simulink model "model"  (R2016a)
(part 9 of 11)

  Dellmensingen___Niederstotzingen_CN_31105067_380000_CN_41389594_380000/RConn3 -- T_41389594_380000;220000;110000_Umspannwerk_Dellmensingen/LConn3 -- 380_kV_CN_26260052_380000_CN_41389594_380000/LConn3 -- _CN_85523877_380000_CN_41389594_380000/RConn3 -- Dellmensingen___Obermooweiler;Dellmensingen_Ost_CN_41389594_380000_CN_31131320_380000/LConn3
  T_130794504_220000;110000_Lübeck/LConn1 -- _CN_130794504_220000_CN_28008024_220000/LConn1
  T_130794504_220000;110000_Lübeck/LConn2 -- _CN_130794504_220000_CN_28008024_220000/LConn2
  T_130794504_220000;110000_Lübeck/LConn3 -- _CN_130794504_220000_CN_28008024_220000/LConn3
  _CN_130794504_220000_CN_28008024_220000/RConn1 -- T_28008024_220000;110000;30000_Hamburg_Nord/LConn1 -- _CN_29344008_220000_CN_28008024_220000/RConn1 -- 202_UW_HH_Nord_UW_Itzehoe_West_CN_60032354_220000_CN_28008024_220000/LConn1 -- _CN_28008024_220000_CN_33148774_220000/LConn1 -- _CN_22720647_220000_CN_28008024_220000/LConn1
  _CN_130794504_220000_CN_28008024_220000/RConn2 -- T_28008024_220000;110000;30000_Hamburg_Nord/LConn2 -- _CN_29344008_220000_CN_28008024_220000/RConn2 -- 202_UW_HH_Nord_UW_Itzehoe_West_CN_60032354_220000_CN_28008024_220000/LConn2 -- _CN_28008024_220000_CN_33148774_220000/LConn2 -- _CN_22720647_220000_CN_28008024_220000/LConn2
  _CN_130794504_220000_CN_28008024_220000/RConn3 -- T_28008024_220000;110000;30000_Hamburg_Nord/LConn3 -- _CN_29344008_220000_CN_28008024_220000/RConn3 -- 202_UW_HH_Nord_UW_Itzehoe_West_CN_60032354_220000_CN_28008024_220000/LConn3 -- _CN_28008024_220000_CN_33148774_220000/LConn3 -- _CN_22720647_220000_CN_28008024_220000/LConn3
  543_CN_32063539_380000_CN_32062544_380000/LConn1 -- T_32063539_380000_Bentwisch_HGÜ/LConn1 -- 546_CN_32063539_380000_CN26389159/LConn1
  543_CN_32063539_380000_CN_32062544_380000/LConn2 -- T_32063539_380000_Bentwisch_HGÜ/LConn2 -- 546_CN_32063539_380000_CN26389159/LConn2
  543_CN_32063539_380000_CN_32062544_380000/LConn3 -- T_32063539_380000_Bentwisch_HGÜ/LConn3 -- 546_CN_32063539_380000_CN26389159/LConn3
  543_CN_32063539_380000_CN_32062544_380000/RConn1 -- T_32062544_380000;220000_Güstrow/LConn1 -- 514_CN_59707532_380000_CN_32062544_380000/LConn1 -- 419_Krümmel___Görries_CN_30040568_380000_CN_32062544_380000/LConn1
  543_CN_32063539_380000_CN_32062544_380000/RConn2 -- T_32062544_380000;220000_Güstrow/LConn2 -- 514_CN_59707532_380000_CN_32062544_380000/LConn2 -- 419_Krümmel___Görries_CN_30040568_380000_CN_32062544_380000/LConn2
  543_CN_32063539_380000_CN_32062544_380000/RConn3 -- T_32062544_380000;220000_Güstrow/LConn3 -- 514_CN_59707532_380000_CN_32062544_380000/LConn3 -- 419_Krümmel___Görries_CN_30040568_380000_CN_32062544_380000/LConn3
  G_26389159_Kraftwerk_Rostock/RConn1 -- 546_CN_32063539_380000_CN26389159/RConn1
  G_26389159_Kraftwerk_Rostock/RConn2 -- 546_CN_32063539_380000_CN26389159/RConn2
  G_26389159_Kraftwerk_Rostock/RConn3 -- 546_CN_32063539_380000_CN26389159/RConn3
  Grafenrheinfeld___Eltmann;Eltmann___Redwitz_CN_24758329_380000_CN_108797675_380000/LConn1 -- T_24758329_380000;110000_Umspannwerk_Eltmann/LConn1 -- Grafenrheinfeld___Eltmann;Eltmann___Redwitz_CN_24758329_380000_CN_28613721_380000/LConn1 -- Grafenrheinfeld___Eltmann;Eltmann___Redwitz_CN_24758329_380000_CN_24757392_380000/LConn1 -- Grafenrheinfeld___Eltmann;Eltmann___Redwitz_CN_24758329_380000_CN_24757833_380000/LConn1 -- Grafenrheinfeld___Eltmann;Eltmann___Redwitz_CN_24758329_380000_CN_24715381_380000/LConn1 -- Grafenrheinfeld___Eltmann;Eltmann___Redwitz_CN_24758329_380000_CN_24705761_380000/LConn1
  Grafenrheinfeld___Eltmann;Eltmann___Redwitz_CN_24758329_380000_CN_108797675_380000/LConn2 -- T_24758329_380000;110000_Umspannwerk_Eltmann/LConn2 -- Grafenrheinfeld___Eltmann;Eltmann___Redwitz_CN_24758329_380000_CN_28613721_380000/LConn2 -- Grafenrheinfeld___Eltmann;Eltmann___Redwitz_CN_24758329_380000_CN_24757392_380000/LConn2 -- Grafenrheinfeld___Eltmann;Eltmann___Redwitz_CN_24758329_380000_CN_24757833_380000/LConn2 -- Grafenrheinfeld___Eltmann;Eltmann___Redwitz_CN_24758329_380000_CN_24715381_380000/LConn2 -- Grafenrheinfeld___Eltmann;Eltmann___Redwitz_CN_24758329_380000_CN_24705761_380000/LConn2
  Grafenrheinfeld___Eltmann;Eltmann___Redwitz_CN_24758329_380000_CN_108797675_380000/LConn3 -- T_24758329_380000;110000_Umspannwerk_Eltmann/LConn3 -- Grafenrheinfeld___Eltmann;Eltmann___Redwitz_CN_24758329_380000_CN_28613721_380000/LConn3 -- Grafenrheinfeld___Eltmann;Eltmann___Redwitz_CN_24758329_380000_CN_24757392_380000/LConn3 -- Grafenrheinfeld___Eltmann;Eltmann___Redwitz_CN_24758329_380000_CN_24757833_380000/LConn3 -- Grafenrheinfeld___Eltmann;Eltmann___Redwitz_CN_24758329_380000_CN_24715381_380000/LConn3 -- Grafenrheinfeld___Eltmann;Eltmann___Redwitz_CN_24758329_380000_CN_24705761_380000/LConn3
  Grafenrheinfeld___Eltmann;Eltmann___Redwitz_CN_24758329_380000_CN_108797675_380000/RConn1 -- T_108797675_380000_Grafenrheinfeld/LConn1 -- _CN_24715381_380000_CN_108797675_380000/LConn1 -- _CN_145002769_380000_CN_108797675_380000/LConn1 -- _CN_24705761_380000_CN_108797675_380000/LConn1 -- AS_GKRO;GKRO_GR_I;DIP_GKB_I;_II_CN_42410916_380000_CN_108797675_380000/LConn1
  Grafenrheinfeld___Eltmann;Eltmann___Redwitz_CN_24758329_380000_CN_108797675_380000/RConn2 -- T_108797675_380000_Grafenrheinfeld/LConn2 -- _CN_24715381_380000_CN_108797675_380000/LConn2 -- _CN_145002769_380000_CN_108797675_380000/LConn2 -- _CN_24705761_380000_CN_108797675_380000/LConn2 -- AS_GKRO;GKRO_GR_I;DIP_GKB_I;_II_CN_42410916_380000_CN_108797675_380000/LConn2
  Grafenrheinfeld___Eltmann;Eltmann___Redwitz_CN_24758329_380000_CN_108797675_380000/RConn3 -- T_108797675_380000_Grafenrheinfeld/LConn3 -- _CN_24715381_380000_CN_108797675_380000/LConn3 -- _CN_145002769_380000_CN_108797675_380000/LConn3 -- _CN_24705761_380000_CN_108797675_380000/LConn3 -- AS_GKRO;GKRO_GR_I;DIP_GKB_I;_II_CN_42410916_380000_CN_108797675_380000/LConn3
  Grafenrheinfeld___Eltmann;Eltmann___Redwitz_CN_24758329_380000_CN_24715381_380000/RConn1 -- T_24715381_380000;220000;110000_Umspannwerk_Bergrheinfeld/LConn1 -- _CN_24715381_380000_CN_108797675_380000/RConn1
  Grafenrheinfeld___Eltmann;Eltmann___Redwitz_CN_24758329_380000_CN_24715381_380000/RConn2 -- T_24715381_380000;220000;110000_Umspannwerk_Bergrheinfeld/LConn2 -- _CN_24715381_380000_CN_108797675_380000/RConn2
  Grafenrheinfeld___Eltmann;Eltmann___Redwitz_CN_24758329_380000_CN_24715381_380000/RConn3 -- T_24715381_380000;220000;110000_Umspannwerk_Bergrheinfeld/LConn3 -- _CN_24715381_380000_CN_108797675_380000/RConn3
  Grafenrheinfeld___Eltmann;Eltmann___Redwitz_CN_24758329_380000_CN_24705761_380000/RConn1 -- T_24705761_380000;220000;110000_Umspannwerk_Raitersaich/LConn1 -- Irsching___Raitersaich_CN_24705761_380000_CN_24768051_380000/LConn1 -- _CN_24705761_380000_CN_108797675_380000/RConn1
  Grafenrheinfeld___Eltmann;Eltmann___Redwitz_CN_24758329_380000_CN_24705761_380000/RConn2 -- T_24705761_380000;220000;110000_Umspannwerk_Raitersaich/LConn2 -- Irsching___Raitersaich_CN_24705761_380000_CN_24768051_380000/LConn2 -- _CN_24705761_380000_CN_108797675_380000/RConn2
  Grafenrheinfeld___Eltmann;Eltmann___Redwitz_CN_24758329_380000_CN_24705761_380000/RConn3 -- T_24705761_380000;220000;110000_Umspannwerk_Raitersaich/LConn3 -- Irsching___Raitersaich_CN_24705761_380000_CN_24768051_380000/LConn3 -- _CN_24705761_380000_CN_108797675_380000/RConn3
  T_28613721_380000;110000_Kriegenbrunn/LConn1 -- Grafenrheinfeld___Eltmann;Eltmann___Redwitz_CN_24758329_380000_CN_28613721_380000/RConn1
  T_28613721_380000;110000_Kriegenbrunn/LConn2 -- Grafenrheinfeld___Eltmann;Eltmann___Redwitz_CN_24758329_380000_CN_28613721_380000/RConn2
  T_28613721_380000;110000_Kriegenbrunn/LConn3 -- Grafenrheinfeld___Eltmann;Eltmann___Redwitz_CN_24758329_380000_CN_28613721_380000/RConn3
  Grafenrheinfeld___Eltmann;Eltmann___Redwitz_CN_24758329_380000_CN_24757392_380000/RConn1 -- T_24757392_380000;110000_Umspannwerk_Redwitz/LConn1 -- Etzenricht___Mechlenreuth___Redwitz_CN_93341407_380000_CN_24757392_380000/LConn1 -- _CN_128277645_380000_CN_24757392_380000/LConn1 -- Altenfeld___Redwitz_CN_149256409_380000_CN_24757392_380000/LConn1
  Grafenrheinfeld___Eltmann;Eltmann___Redwitz_CN_24758329_380000_CN_24757392_380000/RConn2 -- T_24757392_380000;110000_Umspannwerk_Redwitz/LConn2 -- Etzenricht___Mechlenreuth___Redwitz_CN_93341407_380000_CN_24757392_380000/LConn2 -- _CN_128277645_380000_CN_24757392_380000/LConn2 -- Altenfeld___Redwitz_CN_149256409_380000_CN_24757392_380000/LConn2
  Grafenrheinfeld___Eltmann;Eltmann___Redwitz_CN_24758329_380000_CN_24757392_380000/RConn3 -- T_24757392_380000;110000_Umspannwerk_Redwitz/LConn3 -- Etzenricht___Mechlenreuth___Redwitz_CN_93341407_380000_CN_24757392_380000/LConn3 -- _CN_128277645_380000_CN_24757392_380000/LConn3 -- Altenfeld___Redwitz_CN_149256409_380000_CN_24757392_380000/LConn3
  T_24757833_380000_Umspannwerk_Oberhaid/LConn1 -- Grafenrheinfeld___Eltmann;Eltmann___Redwitz_CN_24758329_380000_CN_24757833_380000/RConn1
  T_24757833_380000_Umspannwerk_Oberhaid/LConn2 -- Grafenrheinfeld___Eltmann;Eltmann___Redwitz_CN_24758329_380000_CN_24757833_380000/RConn2
  T_24757833_380000_Umspannwerk_Oberhaid/LConn3 -- Grafenrheinfeld___Eltmann;Eltmann___Redwitz_CN_24758329_380000_CN_24757833_380000/RConn3
  220kV_Itterbach_West_CN_87767098_220000_CN_113546939_220000/LConn1 -- T_87767098_220000_Station_Mettmann/LConn1 -- 220kV_Itterbach_West_CN_87767098_220000_CN_23192640_220000/LConn1 -- 220kV_Itterbach_West_CN_87767098_220000_CN_49577401_220000/LConn1 -- 220kV_Itterbach_West_CN_87767098_220000_CN_23140544_220000/LConn1 -- 220kV_Itterbach_West_CN_87767098_220000_CN_22761839_220000/LConn1
  220kV_Itterbach_West_CN_87767098_220000_CN_113546939_220000/LConn2 -- T_87767098_220000_Station_Mettmann/LConn2 -- 220kV_Itterbach_West_CN_87767098_220000_CN_23192640_220000/LConn2 -- 220kV_Itterbach_West_CN_87767098_220000_CN_49577401_220000/LConn2 -- 220kV_Itterbach_West_CN_87767098_220000_CN_23140544_220000/LConn2 -- 220kV_Itterbach_West_CN_87767098_220000_CN_22761839_220000/LConn2
  220kV_Itterbach_West_CN_87767098_220000_CN_113546939_220000/LConn3 -- T_87767098_220000_Station_Mettmann/LConn3 -- 220kV_Itterbach_West_CN_87767098_220000_CN_23192640_220000/LConn3 -- 220kV_Itterbach_West_CN_87767098_220000_CN_49577401_220000/LConn3 -- 220kV_Itterbach_West_CN_87767098_220000_CN_23140544_220000/LConn3 -- 220kV_Itterbach_West_CN_87767098_220000_CN_22761839_220000/LConn3
  220kV_Itterbach_West_CN_87767098_220000_CN_113546939_220000/RConn1 -- T_113546939_380000;220000_Station_Eiberg/RConn1 -- _CN_66038431_220000_CN_113546939_220000/LConn1 -- L_113546939/LConn1 -- 220kV_Polsum_Süd_CN_29077623_220000_CN_113546939_220000/LConn1
  220kV_Itterbach_West_CN_87767098_220000_CN_113546939_220000/RConn2 -- T_113546939_380000;220000_Station_Eiberg/RConn2 -- _CN_66038431_220000_CN_113546939_220000/LConn2 -- L_113546939/LConn2 -- 220kV_Polsum_Süd_CN_29077623_220000_CN_113546939_220000/LConn2
  220kV_Itterbach_West_CN_87767098_220000_CN_113546939_220000/RConn3 -- T_113546939_380000;220000_Station_Eiberg/RConn3 -- _CN_66038431_220000_CN_113546939_220000/LConn3 -- L_113546939/LConn3 -- 220kV_Polsum_Süd_CN_29077623_220000_CN_113546939_220000/LConn3
  T_23192640_220000;110000_Station_Reisholz/LConn1 -- 220kV_Itterbach_West_CN_87767098_220000_CN_23192640_220000/RConn1
  T_23192640_220000;110000_Station_Reisholz/LConn2 -- 220kV_Itterbach_West_CN_87767098_220000_CN_23192640_220000/RConn2
  T_23192640_220000;110000_Station_Reisholz/LConn3 -- 220kV_Itterbach_West_CN_87767098_220000_CN_23192640_220000/RConn3
  220kV_Itterbach_West_CN_87767098_220000_CN_49577401_220000/RConn1 -- T_49577401_220000;110000_Station_Sankt_Peter_220_kV/LConn1 -- 220_kV_Frixheim_Süd;_Zons_Nord_CN_27919734_220000_CN_49577401_220000/LConn1 -- 220_kV_Frimmersdorf_5e;_Zons_Nord_CN_49577401_220000_CN_31762305_220000/LConn1
  220kV_Itterbach_West_CN_87767098_220000_CN_49577401_220000/RConn2 -- T_49577401_220000;110000_Station_Sankt_Peter_220_kV/LConn2 -- 220_kV_Frixheim_Süd;_Zons_Nord_CN_27919734_220000_CN_49577401_220000/LConn2 -- 220_kV_Frimmersdorf_5e;_Zons_Nord_CN_49577401_220000_CN_31762305_220000/LConn2
  220kV_Itterbach_West_CN_87767098_220000_CN_49577401_220000/RConn3 -- T_49577401_220000;110000_Station_Sankt_Peter_220_kV/LConn3 -- 220_kV_Frixheim_Süd;_Zons_Nord_CN_27919734_220000_CN_49577401_220000/LConn3 -- 220_kV_Frimmersdorf_5e;_Zons_Nord_CN_49577401_220000_CN_31762305_220000/LConn3
  T_23140544_220000;110000_Station_Eller/LConn1 -- 220kV_Itterbach_West_CN_87767098_220000_CN_23140544_220000/RConn1
  T_23140544_220000;110000_Station_Eller/LConn2 -- 220kV_Itterbach_West_CN_87767098_220000_CN_23140544_220000/RConn2
  T_23140544_220000;110000_Station_Eller/LConn3 -- 220kV_Itterbach_West_CN_87767098_220000_CN_23140544_220000/RConn3
  220kV_Itterbach_West_CN_87767098_220000_CN_22761839_220000/RConn1 -- T_22761839_380000;220000;110000_Station_Opladen/RConn1 -- 220_kV_Niederaußem_4d;_Wiesdorf_Ltg__CN_22761839_220000_CN_24839976_220000/LConn1 -- 220_kV_Niederaußem_4d;_Wiesdorf_Ltg__CN_22761839_220000_CN24840439/LConn1 -- 220_kV_Niederaußem_4d;_Wiesdorf_Ltg__CN_22761839_220000_CN_22764922_220000/LConn1 -- 220_kV_Dünnwald_Ost|West_CN_22761839_220000_CN_27871140_220000/LConn1 -- L_22761839/LConn1 -- 220_kV_Bigge_Ost|West_CN_22761839_220000_CN_24667346_220000/LConn1 -- 220_kV_Bigge_Ost|West_CN_22761839_220000_CN_51940126_220000/LConn1 -- 220_kV_Bigge_Ost|West_CN_22761839_220000_CN_132814303_220000/LConn1 -- 220_kV_Niederaußem_4d;_Wiesdorf_Ltg__CN_22761839_220000_CN_22761692_220000/LConn1
  220kV_Itterbach_West_CN_87767098_220000_CN_22761839_220000/RConn2 -- T_22761839_380000;220000;110000_Station_Opladen/RConn2 -- 220_kV_Niederaußem_4d;_Wiesdorf_Ltg__CN_22761839_220000_CN_24839976_220000/LConn2 -- 220_kV_Niederaußem_4d;_Wiesdorf_Ltg__CN_22761839_220000_CN24840439/LConn2 -- 220_kV_Niederaußem_4d;_Wiesdorf_Ltg__CN_22761839_220000_CN_22764922_220000/LConn2 -- 220_kV_Dünnwald_Ost|West_CN_22761839_220000_CN_27871140_220000/LConn2 -- L_22761839/LConn2 -- 220_kV_Bigge_Ost|West_CN_22761839_220000_CN_24667346_220000/LConn2 -- 220_kV_Bigge_Ost|West_CN_22761839_220000_CN_51940126_220000/LConn2 -- 220_kV_Bigge_Ost|West_CN_22761839_220000_CN_132814303_220000/LConn2 -- 220_kV_Niederaußem_4d;_Wiesdorf_Ltg__CN_22761839_220000_CN_22761692_220000/LConn2
  220kV_Itterbach_West_CN_87767098_220000_CN_22761839_220000/RConn3 -- T_22761839_380000;220000;110000_Station_Opladen/RConn3 -- 220_kV_Niederaußem_4d;_Wiesdorf_Ltg__CN_22761839_220000_CN_24839976_220000/LConn3 -- 220_kV_Niederaußem_4d;_Wiesdorf_Ltg__CN_22761839_220000_CN24840439/LConn3 -- 220_kV_Niederaußem_4d;_Wiesdorf_Ltg__CN_22761839_220000_CN_22764922_220000/LConn3 -- 220_kV_Dünnwald_Ost|West_CN_22761839_220000_CN_27871140_220000/LConn3 -- L_22761839/LConn3 -- 220_kV_Bigge_Ost|West_CN_22761839_220000_CN_24667346_220000/LConn3 -- 220_kV_Bigge_Ost|West_CN_22761839_220000_CN_51940126_220000/LConn3 -- 220_kV_Bigge_Ost|West_CN_22761839_220000_CN_132814303_220000/LConn3 -- 220_kV_Niederaußem_4d;_Wiesdorf_Ltg__CN_22761839_220000_CN_22761692_220000/LConn3
  _CN_88916034_380000_CN_35954395_380000/LConn1 -- T_88916034_380000;220000_Lastverteilung_Schaltanlage_Kühmoos/LConn1 -- _CN_88916034_380000_CN_25306752_380000/LConn1 -- _CN_88916034_380000_CN_31367940_380000/LConn1 -- _CN_88916034_380000_CN_202865177_380000/LConn1 -- _CN_88916034_380000_CN_88901626_380000/LConn1 -- _CN_88916034_380000_CN_242756113_380000/LConn1 -- _CN_88916034_380000_CN_152261133_380000/LConn1 -- _CN_88916034_380000_CN_42736239_380000/LConn1 -- _CN_88916034_380000_CN_42049947_380000/LConn1
  _CN_88916034_380000_CN_35954395_380000/LConn2 -- T_88916034_380000;220000_Lastverteilung_Schaltanlage_Kühmoos/LConn2 -- _CN_88916034_380000_CN_25306752_380000/LConn2 -- _CN_88916034_380000_CN_31367940_380000/LConn2 -- _CN_88916034_380000_CN_202865177_380000/LConn2 -- _CN_88916034_380000_CN_88901626_380000/LConn2 -- _CN_88916034_380000_CN_242756113_380000/LConn2 -- _CN_88916034_380000_CN_152261133_380000/LConn2 -- _CN_88916034_380000_CN_42736239_380000/LConn2 -- _CN_88916034_380000_CN_42049947_380000/LConn2
  _CN_88916034_380000_CN_35954395_380000/LConn3 -- T_88916034_380000;220000_Lastverteilung_Schaltanlage_Kühmoos/LConn3 -- _CN_88916034_380000_CN_25306752_380000/LConn3 -- _CN_88916034_380000_CN_31367940_380000/LConn3 -- _CN_88916034_380000_CN_202865177_380000/LConn3 -- _CN_88916034_380000_CN_88901626_380000/LConn3 -- _CN_88916034_380000_CN_242756113_380000/LConn3 -- _CN_88916034_380000_CN_152261133_380000/LConn3 -- _CN_88916034_380000_CN_42736239_380000/LConn3 -- _CN_88916034_380000_CN_42049947_380000/LConn3
  T_35954395_380000;110000_Umspannwerk_Trossingen/LConn1 -- _CN_88916034_380000_CN_35954395_380000/RConn1
  T_35954395_380000;110000_Umspannwerk_Trossingen/LConn2 -- _CN_88916034_380000_CN_35954395_380000/RConn2
  T_35954395_380000;110000_Umspannwerk_Trossingen/LConn3 -- _CN_88916034_380000_CN_35954395_380000/RConn3
  _CN_88916034_380000_CN_42736239_380000/RConn1 -- T_42736239_380000_EnBW_Umspannwerk_Engstlatt/LConn1 -- PULVE_OBJTT_ENGST_380_kV;_OBJTT_ENGST_380_kV;_TRSNG_WDLNG_220_kV_CN_42736239_380000_CN_26814283_380000/LConn1
  _CN_88916034_380000_CN_42736239_380000/RConn2 -- T_42736239_380000_EnBW_Umspannwerk_Engstlatt/LConn2 -- PULVE_OBJTT_ENGST_380_kV;_OBJTT_ENGST_380_kV;_TRSNG_WDLNG_220_kV_CN_42736239_380000_CN_26814283_380000/LConn2
  _CN_88916034_380000_CN_42736239_380000/RConn3 -- T_42736239_380000_EnBW_Umspannwerk_Engstlatt/LConn3 -- PULVE_OBJTT_ENGST_380_kV;_OBJTT_ENGST_380_kV;_TRSNG_WDLNG_220_kV_CN_42736239_380000_CN_26814283_380000/LConn3
  T_42049947_380000;110000_Umspannwerk_Villingen/LConn1 -- _CN_88916034_380000_CN_42049947_380000/RConn1
  T_42049947_380000;110000_Umspannwerk_Villingen/LConn2 -- _CN_88916034_380000_CN_42049947_380000/RConn2
  T_42049947_380000;110000_Umspannwerk_Villingen/LConn3 -- _CN_88916034_380000_CN_42049947_380000/RConn3
  T_88901626_380000;110000_Schwörstadt/LConn1 -- _CN_88916034_380000_CN_88901626_380000/RConn1
  T_88901626_380000;110000_Schwörstadt/LConn2 -- _CN_88916034_380000_CN_88901626_380000/RConn2
  T_88901626_380000;110000_Schwörstadt/LConn3 -- _CN_88916034_380000_CN_88901626_380000/RConn3
  T_242756113_380000;220000;110000_380_kV_Umspannwerk_Eichstetten/LConn1 -- _CN_88916034_380000_CN_242756113_380000/RConn1
  T_242756113_380000;220000;110000_380_kV_Umspannwerk_Eichstetten/LConn2 -- _CN_88916034_380000_CN_242756113_380000/RConn2
  T_242756113_380000;220000;110000_380_kV_Umspannwerk_Eichstetten/LConn3 -- _CN_88916034_380000_CN_242756113_380000/RConn3
  _CN_88916034_380000_CN_152261133_380000/RConn1 -- T_152261133_380000;220000;110000_Karlsruhe_Daxlanden/LConn1 -- _CN_152261133_380000_CN_149987048_380000/LConn1 -- _CN_152261133_380000_CN_54359256_380000/LConn1 -- _CN_152261133_380000_CN_152018146_380000/LConn1 -- _CN_152261133_380000_CN161909939/LConn1 -- 7563_CN_152261133_380000_CN_272646943_380000/LConn1 -- 7564_CN_152261133_380000_CN_194446360_380000/LConn1
  _CN_88916034_380000_CN_152261133_380000/RConn2 -- T_152261133_380000;220000;110000_Karlsruhe_Daxlanden/LConn2 -- _CN_152261133_380000_CN_149987048_380000/LConn2 -- _CN_152261133_380000_CN_54359256_380000/LConn2 -- _CN_152261133_380000_CN_152018146_380000/LConn2 -- _CN_152261133_380000_CN161909939/LConn2 -- 7563_CN_152261133_380000_CN_272646943_380000/LConn2 -- 7564_CN_152261133_380000_CN_194446360_380000/LConn2
  _CN_88916034_380000_CN_152261133_380000/RConn3 -- T_152261133_380000;220000;110000_Karlsruhe_Daxlanden/LConn3 -- _CN_152261133_380000_CN_149987048_380000/LConn3 -- _CN_152261133_380000_CN_54359256_380000/LConn3 -- _CN_152261133_380000_CN_152018146_380000/LConn3 -- _CN_152261133_380000_CN161909939/LConn3 -- 7563_CN_152261133_380000_CN_272646943_380000/LConn3 -- 7564_CN_152261133_380000_CN_194446360_380000/LConn3
  _CN_88916034_380000_CN_25306752_380000/RConn1 -- T_25306752_380000;220000;110000_Umspannwerk_Herbertingen/LConn1 -- Herbertingen___Grünkraut_CN_25306752_380000_CN_31131325_380000/LConn1
  _CN_88916034_380000_CN_25306752_380000/RConn2 -- T_25306752_380000;220000;110000_Umspannwerk_Herbertingen/LConn2 -- Herbertingen___Grünkraut_CN_25306752_380000_CN_31131325_380000/LConn2
  _CN_88916034_380000_CN_25306752_380000/RConn3 -- T_25306752_380000;220000;110000_Umspannwerk_Herbertingen/LConn3 -- Herbertingen___Grünkraut_CN_25306752_380000_CN_31131325_380000/LConn3
  T_31367940_380000;220000;110000_Tiengen/LConn1 -- _CN_88916034_380000_CN_31367940_380000/RConn1
  T_31367940_380000;220000;110000_Tiengen/LConn2 -- _CN_88916034_380000_CN_31367940_380000/RConn2
  T_31367940_380000;220000;110000_Tiengen/LConn3 -- _CN_88916034_380000_CN_31367940_380000/RConn3
  _CN_88916034_220000_CN_202865176_220000/LConn1 -- T_88916034_380000;220000_Lastverteilung_Schaltanlage_Kühmoos/RConn1 -- L_88916034/LConn1
  _CN_88916034_220000_CN_202865176_220000/LConn2 -- T_88916034_380000;220000_Lastverteilung_Schaltanlage_Kühmoos/RConn2 -- L_88916034/LConn2
  _CN_88916034_220000_CN_202865176_220000/LConn3 -- T_88916034_380000;220000_Lastverteilung_Schaltanlage_Kühmoos/RConn3 -- L_88916034/LConn3
  _CN_88916034_220000_CN_202865176_220000/RConn1 -- T_202865176_220000_/LConn1 -- Öldruckkabel_CN_202865176_220000_CN129989100/LConn1
  _CN_88916034_220000_CN_202865176_220000/RConn2 -- T_202865176_220000_/LConn2 -- Öldruckkabel_CN_202865176_220000_CN129989100/LConn2
  _CN_88916034_220000_CN_202865176_220000/RConn3 -- T_202865176_220000_/LConn3 -- Öldruckkabel_CN_202865176_220000_CN129989100/LConn3
  T_202865177_380000_Kabelanfang_PSP_Wehr/LConn1 -- _CN_88916034_380000_CN_202865177_380000/RConn1
  T_202865177_380000_Kabelanfang_PSP_Wehr/LConn2 -- _CN_88916034_380000_CN_202865177_380000/RConn2
  T_202865177_380000_Kabelanfang_PSP_Wehr/LConn3 -- _CN_88916034_380000_CN_202865177_380000/RConn3
  _CN_32151621_220000_CN_39011884_220000/LConn1 -- T_32151621_220000;110000_220_kV_Umspannwerk_Kuppenheim/LConn1 -- _CN_32151621_220000_CN_146962222_220000/LConn1 -- _CN_32151621_220000_CN_152261133_220000/LConn1
  _CN_32151621_220000_CN_39011884_220000/LConn2 -- T_32151621_220000;110000_220_kV_Umspannwerk_Kuppenheim/LConn2 -- _CN_32151621_220000_CN_146962222_220000/LConn2 -- _CN_32151621_220000_CN_152261133_220000/LConn2
  _CN_32151621_220000_CN_39011884_220000/LConn3 -- T_32151621_220000;110000_220_kV_Umspannwerk_Kuppenheim/LConn3 -- _CN_32151621_220000_CN_146962222_220000/LConn3 -- _CN_32151621_220000_CN_152261133_220000/LConn3
  T_39011884_220000;110000_Bühl/LConn1 -- _CN_32151621_220000_CN_39011884_220000/RConn1
  T_39011884_220000;110000_Bühl/LConn2 -- _CN_32151621_220000_CN_39011884_220000/RConn2
  T_39011884_220000;110000_Bühl/LConn3 -- _CN_32151621_220000_CN_39011884_220000/RConn3
  _CN_32151621_220000_CN_146962222_220000/RConn1 -- T_146962222_220000;110000_Umspannwerk_Weier/LConn1 -- _CN_87653464_220000_CN_146962222_220000/LConn1
  _CN_32151621_220000_CN_146962222_220000/RConn2 -- T_146962222_220000;110000_Umspannwerk_Weier/LConn2 -- _CN_87653464_220000_CN_146962222_220000/LConn2
  _CN_32151621_220000_CN_146962222_220000/RConn3 -- T_146962222_220000;110000_Umspannwerk_Weier/LConn3 -- _CN_87653464_220000_CN_146962222_220000/LConn3
  _CN_32151621_220000_CN_152261133_220000/RConn1 -- T_152261133_380000;220000;110000_Karlsruhe_Daxlanden/RConn1 -- Daxlanden___Mühlburg_CN_32731290_220000_CN_152261133_220000/LConn1 -- _CN_152261133_220000_CN_207248812_220000/RConn1 -- _CN_152261133_220000_CN_163093653_220000/LConn1 -- _CN_152261133_220000_CN_160929097_220000/LConn1 -- _CN_152261133_220000_CN_154729020_220000/LConn1 -- _CN_152261133_220000_CN_32966636_220000/LConn1 -- _CN_152261133_220000_CN_32725957_220000/LConn1 -- L_152261133/LConn1 -- 220_kV_Kondelwald;_220kV_Wengerohr_CN_66764943_220000_CN_152261133_220000/LConn1
  _CN_32151621_220000_CN_152261133_220000/RConn2 -- T_152261133_380000;220000;110000_Karlsruhe_Daxlanden/RConn2 -- Daxlanden___Mühlburg_CN_32731290_220000_CN_152261133_220000/LConn2 -- _CN_152261133_220000_CN_207248812_220000/RConn2 -- _CN_152261133_220000_CN_163093653_220000/LConn2 -- _CN_152261133_220000_CN_160929097_220000/LConn2 -- _CN_152261133_220000_CN_154729020_220000/LConn2 -- _CN_152261133_220000_CN_32966636_220000/LConn2 -- _CN_152261133_220000_CN_32725957_220000/LConn2 -- L_152261133/LConn2 -- 220_kV_Kondelwald;_220kV_Wengerohr_CN_66764943_220000_CN_152261133_220000/LConn2
  _CN_32151621_220000_CN_152261133_220000/RConn3 -- T_152261133_380000;220000;110000_Karlsruhe_Daxlanden/RConn3 -- Daxlanden___Mühlburg_CN_32731290_220000_CN_152261133_220000/LConn3 -- _CN_152261133_220000_CN_207248812_220000/RConn3 -- _CN_152261133_220000_CN_163093653_220000/LConn3 -- _CN_152261133_220000_CN_160929097_220000/LConn3 -- _CN_152261133_220000_CN_154729020_220000/LConn3 -- _CN_152261133_220000_CN_32966636_220000/LConn3 -- _CN_152261133_220000_CN_32725957_220000/LConn3 -- L_152261133/LConn3 -- 220_kV_Kondelwald;_220kV_Wengerohr_CN_66764943_220000_CN_152261133_220000/LConn3
  Irsching___Ottenhofen;Oberbachern___Ottenhofen_CN_26245195_380000_CN29122363/LConn1 -- T_26245195_380000;220000_Umspannwerk_Ottenhofen/LConn1 -- Irsching___Ottenhofen;Oberbachern___Ottenhofen_CN_26245195_380000_CN_18629425_380000/LConn1 -- Isar___Ottenhofen_CN_26245195_380000_CN23802422/LConn1 -- OH_FO_CN_26245195_380000_CN_5404079_380000/LConn1
  Irsching___Ottenhofen;Oberbachern___Ottenhofen_CN_26245195_380000_CN29122363/LConn2 -- T_26245195_380000;220000_Umspannwerk_Ottenhofen/LConn2 -- Irsching___Ottenhofen;Oberbachern___Ottenhofen_CN_26245195_380000_CN_18629425_380000/LConn2 -- Isar___Ottenhofen_CN_26245195_380000_CN23802422/LConn2 -- OH_FO_CN_26245195_380000_CN_5404079_380000/LConn2
  Irsching___Ottenhofen;Oberbachern___Ottenhofen_CN_26245195_380000_CN29122363/LConn3 -- T_26245195_380000;220000_Umspannwerk_Ottenhofen/LConn3 -- Irsching___Ottenhofen;Oberbachern___Ottenhofen_CN_26245195_380000_CN_18629425_380000/LConn3 -- Isar___Ottenhofen_CN_26245195_380000_CN23802422/LConn3 -- OH_FO_CN_26245195_380000_CN_5404079_380000/LConn3
  Irsching___Ottenhofen;Oberbachern___Ottenhofen_CN_26245195_380000_CN29122363/RConn1 -- G_29122363_Kraftwerk_Irsching/RConn1 -- Neufinsing___Zolling_CN_24158385_220000_CN29122363/LConn1 -- _CN_137602559_220000_CN29122363/LConn1
  Irsching___Ottenhofen;Oberbachern___Ottenhofen_CN_26245195_380000_CN29122363/RConn2 -- G_29122363_Kraftwerk_Irsching/RConn2 -- Neufinsing___Zolling_CN_24158385_220000_CN29122363/LConn2 -- _CN_137602559_220000_CN29122363/LConn2
  Irsching___Ottenhofen;Oberbachern___Ottenhofen_CN_26245195_380000_CN29122363/RConn3 -- G_29122363_Kraftwerk_Irsching/RConn3 -- Neufinsing___Zolling_CN_24158385_220000_CN29122363/LConn3 -- _CN_137602559_220000_CN29122363/LConn3
  Irsching___Ottenhofen;Oberbachern___Ottenhofen_CN_26245195_380000_CN_18629425_380000/RConn1 -- T_18629425_380000;220000;110000_Umspannwerk_Oberbachern/LConn1 -- MEI_OBA_CN_24652261_380000_CN_18629425_380000/LConn1 -- OBA___MZ_CN_18629425_380000_CN_23907283_380000/LConn1
  Irsching___Ottenhofen;Oberbachern___Ottenhofen_CN_26245195_380000_CN_18629425_380000/RConn2 -- T_18629425_380000;220000;110000_Umspannwerk_Oberbachern/LConn2 -- MEI_OBA_CN_24652261_380000_CN_18629425_380000/LConn2 -- OBA___MZ_CN_18629425_380000_CN_23907283_380000/LConn2
  Irsching___Ottenhofen;Oberbachern___Ottenhofen_CN_26245195_380000_CN_18629425_380000/RConn3 -- T_18629425_380000;220000;110000_Umspannwerk_Oberbachern/LConn3 -- MEI_OBA_CN_24652261_380000_CN_18629425_380000/LConn3 -- OBA___MZ_CN_18629425_380000_CN_23907283_380000/LConn3
  Isar___Ottenhofen_CN_26245195_380000_CN23802422/RConn1 -- G_23802422_Kernkraftwerk_Isar/RConn1 -- _CN_77697810_380000_CN23802422/LConn1
  Isar___Ottenhofen_CN_26245195_380000_CN23802422/RConn2 -- G_23802422_Kernkraftwerk_Isar/RConn2 -- _CN_77697810_380000_CN23802422/LConn2
  Isar___Ottenhofen_CN_26245195_380000_CN23802422/RConn3 -- G_23802422_Kernkraftwerk_Isar/RConn3 -- _CN_77697810_380000_CN23802422/LConn3
  _CN_26245195_220000_CN_24158385_220000/LConn1 -- T_26245195_380000;220000_Umspannwerk_Ottenhofen/RConn1 -- L_26245195/LConn1
  _CN_26245195_220000_CN_24158385_220000/LConn2 -- T_26245195_380000;220000_Umspannwerk_Ottenhofen/RConn2 -- L_26245195/LConn2
  _CN_26245195_220000_CN_24158385_220000/LConn3 -- T_26245195_380000;220000_Umspannwerk_Ottenhofen/RConn3 -- L_26245195/LConn3
  _CN_26245195_220000_CN_24158385_220000/RConn1 -- T_24158385_220000;110000_Umspannwerk_Neufinsing/LConn1 -- Oberbachern___Neufinsing_CN_24158385_220000_CN_18629425_220000/LConn1 -- Neufinsing___Zolling_CN_24158385_220000_CN_133342285_220000/LConn1 -- Neufinsing___Zolling_CN_24158385_220000_CN29122363/RConn1 -- _CN_24158385_220000_CN_75865676_220000/LConn1
  _CN_26245195_220000_CN_24158385_220000/RConn2 -- T_24158385_220000;110000_Umspannwerk_Neufinsing/LConn2 -- Oberbachern___Neufinsing_CN_24158385_220000_CN_18629425_220000/LConn2 -- Neufinsing___Zolling_CN_24158385_220000_CN_133342285_220000/LConn2 -- Neufinsing___Zolling_CN_24158385_220000_CN29122363/RConn2 -- _CN_24158385_220000_CN_75865676_220000/LConn2
  _CN_26245195_220000_CN_24158385_220000/RConn3 -- T_24158385_220000;110000_Umspannwerk_Neufinsing/LConn3 -- Oberbachern___Neufinsing_CN_24158385_220000_CN_18629425_220000/LConn3 -- Neufinsing___Zolling_CN_24158385_220000_CN_133342285_220000/LConn3 -- Neufinsing___Zolling_CN_24158385_220000_CN29122363/RConn3 -- _CN_24158385_220000_CN_75865676_220000/LConn3
  T_5404079_380000;110000_Föhring/LConn1 -- OH_FO_CN_26245195_380000_CN_5404079_380000/RConn1
  T_5404079_380000;110000_Föhring/LConn2 -- OH_FO_CN_26245195_380000_CN_5404079_380000/RConn2
  T_5404079_380000;110000_Föhring/LConn3 -- OH_FO_CN_26245195_380000_CN_5404079_380000/RConn3
  220_kV_Merheim_Ost|West_CN_29374542_220000_CN_27871140_220000/LConn1 -- T_29374542_220000;110000_Station_Gremberghoven/LConn1 -- 220_kV_Gremberghoven_Ost|West_CN_29374542_220000_CN_22767509_220000/LConn1 -- 220_kV_Gremberghoven_Ost|West_CN_29374542_220000_CN_22796434_220000/LConn1
  220_kV_Merheim_Ost|West_CN_29374542_220000_CN_27871140_220000/LConn2 -- T_29374542_220000;110000_Station_Gremberghoven/LConn2 -- 220_kV_Gremberghoven_Ost|West_CN_29374542_220000_CN_22767509_220000/LConn2 -- 220_kV_Gremberghoven_Ost|West_CN_29374542_220000_CN_22796434_220000/LConn2
  220_kV_Merheim_Ost|West_CN_29374542_220000_CN_27871140_220000/LConn3 -- T_29374542_220000;110000_Station_Gremberghoven/LConn3 -- 220_kV_Gremberghoven_Ost|West_CN_29374542_220000_CN_22767509_220000/LConn3 -- 220_kV_Gremberghoven_Ost|West_CN_29374542_220000_CN_22796434_220000/LConn3
  220_kV_Merheim_Ost|West_CN_29374542_220000_CN_27871140_220000/RConn1 -- T_27871140_220000_Station_Dünnwald/LConn1 -- 220_kV_Dünnwald_Ost|West_CN_22761839_220000_CN_27871140_220000/RConn1
  220_kV_Merheim_Ost|West_CN_29374542_220000_CN_27871140_220000/RConn2 -- T_27871140_220000_Station_Dünnwald/LConn2 -- 220_kV_Dünnwald_Ost|West_CN_22761839_220000_CN_27871140_220000/RConn2
  220_kV_Merheim_Ost|West_CN_29374542_220000_CN_27871140_220000/RConn3 -- T_27871140_220000_Station_Dünnwald/LConn3 -- 220_kV_Dünnwald_Ost|West_CN_22761839_220000_CN_27871140_220000/RConn3
  220_kV_Gremberghoven_Ost|West_CN_29374542_220000_CN_22767509_220000/RConn1 -- T_22767509_220000;110000_Station_Siegburg/LConn1 -- 220_kV_Leuscheid_Nord+Süd_CN_152403632_220000_CN_22767509_220000/LConn1 -- 220_kV_Troisdorf_West_CN_22766160_220000_CN_22767509_220000/LConn1
  220_kV_Gremberghoven_Ost|West_CN_29374542_220000_CN_22767509_220000/RConn2 -- T_22767509_220000;110000_Station_Siegburg/LConn2 -- 220_kV_Leuscheid_Nord+Süd_CN_152403632_220000_CN_22767509_220000/LConn2 -- 220_kV_Troisdorf_West_CN_22766160_220000_CN_22767509_220000/LConn2
  220_kV_Gremberghoven_Ost|West_CN_29374542_220000_CN_22767509_220000/RConn3 -- T_22767509_220000;110000_Station_Siegburg/LConn3 -- 220_kV_Leuscheid_Nord+Süd_CN_152403632_220000_CN_22767509_220000/LConn3 -- 220_kV_Troisdorf_West_CN_22766160_220000_CN_22767509_220000/LConn3
  T_22796434_220000;110000_Station_Stockem/LConn1 -- 220_kV_Gremberghoven_Ost|West_CN_29374542_220000_CN_22796434_220000/RConn1
  T_22796434_220000;110000_Station_Stockem/LConn2 -- 220_kV_Gremberghoven_Ost|West_CN_29374542_220000_CN_22796434_220000/RConn2
  T_22796434_220000;110000_Station_Stockem/LConn3 -- 220_kV_Gremberghoven_Ost|West_CN_29374542_220000_CN_22796434_220000/RConn3
  _CN_29472852_220000_CN_114319248_220000/LConn1 -- T_29472852_220000;110000_Station_Ibbenbüren/LConn1 -- 110kV_Velpe_Nord_CN_29472852_220000_CN_61918154_220000/LConn1 -- 110kV_Velpe_Nord_CN_29472852_220000_CN_29077623_220000/LConn1 -- _CN_29472852_220000_CN_37764852_220000/LConn1 -- 110kV_Velpe_Nord_CN_29472852_220000_CN_42861703_220000/LConn1 -- 110kV_Velpe_Nord_CN_29472852_220000_CN_42507488_220000/LConn1
  _CN_29472852_220000_CN_114319248_220000/LConn2 -- T_29472852_220000;110000_Station_Ibbenbüren/LConn2 -- 110kV_Velpe_Nord_CN_29472852_220000_CN_61918154_220000/LConn2 -- 110kV_Velpe_Nord_CN_29472852_220000_CN_29077623_220000/LConn2 -- _CN_29472852_220000_CN_37764852_220000/LConn2 -- 110kV_Velpe_Nord_CN_29472852_220000_CN_42861703_220000/LConn2 -- 110kV_Velpe_Nord_CN_29472852_220000_CN_42507488_220000/LConn2
  _CN_29472852_220000_CN_114319248_220000/LConn3 -- T_29472852_220000;110000_Station_Ibbenbüren/LConn3 -- 110kV_Velpe_Nord_CN_29472852_220000_CN_61918154_220000/LConn3 -- 110kV_Velpe_Nord_CN_29472852_220000_CN_29077623_220000/LConn3 -- _CN_29472852_220000_CN_37764852_220000/LConn3 -- 110kV_Velpe_Nord_CN_29472852_220000_CN_42861703_220000/LConn3 -- 110kV_Velpe_Nord_CN_29472852_220000_CN_42507488_220000/LConn3
  _CN_29472852_220000_CN_114319248_220000/RConn1 -- T_114319248_380000;220000;110000_Station_Westerkappeln/RConn1 -- _CN_33411203_220000_CN_114319248_220000/LConn1 -- 220kV_Ibbenbüren_B_CN_114319248_220000_CN196878039/LConn1 -- L_114319248/LConn1
  _CN_29472852_220000_CN_114319248_220000/RConn2 -- T_114319248_380000;220000;110000_Station_Westerkappeln/RConn2 -- _CN_33411203_220000_CN_114319248_220000/LConn2 -- 220kV_Ibbenbüren_B_CN_114319248_220000_CN196878039/LConn2 -- L_114319248/LConn2
  _CN_29472852_220000_CN_114319248_220000/RConn3 -- T_114319248_380000;220000;110000_Station_Westerkappeln/RConn3 -- _CN_33411203_220000_CN_114319248_220000/LConn3 -- 220kV_Ibbenbüren_B_CN_114319248_220000_CN196878039/LConn3 -- L_114319248/LConn3
  _CN_29472852_220000_CN_37764852_220000/RConn1 -- T_37764852_220000;110000_Station_Lüstringen/LConn1 -- _CN_33411203_220000_CN_37764852_220000/LConn1 -- _CN_26383042_220000_CN_37764852_220000/LConn1
  _CN_29472852_220000_CN_37764852_220000/RConn2 -- T_37764852_220000;110000_Station_Lüstringen/LConn2 -- _CN_33411203_220000_CN_37764852_220000/LConn2 -- _CN_26383042_220000_CN_37764852_220000/LConn2
  _CN_29472852_220000_CN_37764852_220000/RConn3 -- T_37764852_220000;110000_Station_Lüstringen/LConn3 -- _CN_33411203_220000_CN_37764852_220000/LConn3 -- _CN_26383042_220000_CN_37764852_220000/LConn3
  110kV_Velpe_Nord_CN_29472852_220000_CN_42861703_220000/RConn1 -- T_42861703_220000_Amelsbüren/LConn1 -- _CN_111973179_220000_CN_42861703_220000/LConn1
  110kV_Velpe_Nord_CN_29472852_220000_CN_42861703_220000/RConn2 -- T_42861703_220000_Amelsbüren/LConn2 -- _CN_111973179_220000_CN_42861703_220000/LConn2
  110kV_Velpe_Nord_CN_29472852_220000_CN_42861703_220000/RConn3 -- T_42861703_220000_Amelsbüren/LConn3 -- _CN_111973179_220000_CN_42861703_220000/LConn3
  110kV_Velpe_Nord_CN_29472852_220000_CN_42507488_220000/RConn1 -- T_42507488_380000;220000;110000_Station_Gersteinwerk/RConn1 -- _CN_24414688_220000_CN_42507488_220000/LConn1 -- 220kV_Cappenberg_Nord+Elmenhorst_Süd_CN_138877959_220000_CN_42507488_220000/LConn1 -- 220kV_Gersteinwerk_I2_CN_42507488_220000_CN33883956/LConn1 -- L_42507488/LConn1
  110kV_Velpe_Nord_CN_29472852_220000_CN_42507488_220000/RConn2 -- T_42507488_380000;220000;110000_Station_Gersteinwerk/RConn2 -- _CN_24414688_220000_CN_42507488_220000/LConn2 -- 220kV_Cappenberg_Nord+Elmenhorst_Süd_CN_138877959_220000_CN_42507488_220000/LConn2 -- 220kV_Gersteinwerk_I2_CN_42507488_220000_CN33883956/LConn2 -- L_42507488/LConn2
  110kV_Velpe_Nord_CN_29472852_220000_CN_42507488_220000/RConn3 -- T_42507488_380000;220000;110000_Station_Gersteinwerk/RConn3 -- _CN_24414688_220000_CN_42507488_220000/LConn3 -- 220kV_Cappenberg_Nord+Elmenhorst_Süd_CN_138877959_220000_CN_42507488_220000/LConn3 -- 220kV_Gersteinwerk_I2_CN_42507488_220000_CN33883956/LConn3 -- L_42507488/LConn3
  110kV_Velpe_Nord_CN_29472852_220000_CN_61918154_220000/RConn1 -- T_61918154_380000;220000;110000_Hanekenfähr/RConn1 -- 220kV_Benteler_CN_118928165_220000_CN_61918154_220000/LConn1 -- L_61918154/LConn1
  110kV_Velpe_Nord_CN_29472852_220000_CN_61918154_220000/RConn2 -- T_61918154_380000;220000;110000_Hanekenfähr/RConn2 -- 220kV_Benteler_CN_118928165_220000_CN_61918154_220000/LConn2 -- L_61918154/LConn2
  110kV_Velpe_Nord_CN_29472852_220000_CN_61918154_220000/RConn3 -- T_61918154_380000;220000;110000_Hanekenfähr/RConn3 -- 220kV_Benteler_CN_118928165_220000_CN_61918154_220000/LConn3 -- L_61918154/LConn3
  110kV_Velpe_Nord_CN_29472852_220000_CN_29077623_220000/RConn1 -- T_29077623_380000;220000;110000_Station_Kusenhorst/RConn1 -- 220kV_Polsum_Süd_CN_29077623_220000_CN_23022100_220000/LConn1 -- 220kV_Polsum_Süd_CN_29077623_220000_CN_38584673_220000/LConn1 -- 220kV_Polsum_Süd_CN_29077623_220000_CN_22944791_220000/LConn1 -- 220kV_Polsum_Süd_CN_29077623_220000_CN_28452784_220000/LConn1 -- 220kV_Polsum_Süd_CN_29077623_220000_CN_68549340_220000/LConn1 -- 220kV_Polsum_Süd_CN_29077623_220000_CN_29282738_220000/LConn1 -- 220kV_Polsum_Süd_CN_29077623_220000_CN_113546939_220000/RConn1 -- 220kV_Polsum_Süd_CN_29077623_220000_CN25649285/LConn1 -- L_29077623/LConn1
  110kV_Velpe_Nord_CN_29472852_220000_CN_29077623_220000/RConn2 -- T_29077623_380000;220000;110000_Station_Kusenhorst/RConn2 -- 220kV_Polsum_Süd_CN_29077623_220000_CN_23022100_220000/LConn2 -- 220kV_Polsum_Süd_CN_29077623_220000_CN_38584673_220000/LConn2 -- 220kV_Polsum_Süd_CN_29077623_220000_CN_22944791_220000/LConn2 -- 220kV_Polsum_Süd_CN_29077623_220000_CN_28452784_220000/LConn2 -- 220kV_Polsum_Süd_CN_29077623_220000_CN_68549340_220000/LConn2 -- 220kV_Polsum_Süd_CN_29077623_220000_CN_29282738_220000/LConn2 -- 220kV_Polsum_Süd_CN_29077623_220000_CN_113546939_220000/RConn2 -- 220kV_Polsum_Süd_CN_29077623_220000_CN25649285/LConn2 -- L_29077623/LConn2
  110kV_Velpe_Nord_CN_29472852_220000_CN_29077623_220000/RConn3 -- T_29077623_380000;220000;110000_Station_Kusenhorst/RConn3 -- 220kV_Polsum_Süd_CN_29077623_220000_CN_23022100_220000/LConn3 -- 220kV_Polsum_Süd_CN_29077623_220000_CN_38584673_220000/LConn3 -- 220kV_Polsum_Süd_CN_29077623_220000_CN_22944791_220000/LConn3 -- 220kV_Polsum_Süd_CN_29077623_220000_CN_28452784_220000/LConn3 -- 220kV_Polsum_Süd_CN_29077623_220000_CN_68549340_220000/LConn3 -- 220kV_Polsum_Süd_CN_29077623_220000_CN_29282738_220000/LConn3 -- 220kV_Polsum_Süd_CN_29077623_220000_CN_113546939_220000/RConn3 -- 220kV_Polsum_Süd_CN_29077623_220000_CN25649285/LConn3 -- L_29077623/LConn3
  T_202164315_380000_KW_Heyden/LConn1 -- Leitung_3016_CN_202164315_380000_CN_24604789_380000/LConn1
  T_202164315_380000_KW_Heyden/LConn2 -- Leitung_3016_CN_202164315_380000_CN_24604789_380000/LConn2
  T_202164315_380000_KW_Heyden/LConn3 -- Leitung_3016_CN_202164315_380000_CN_24604789_380000/LConn3
  Leitung_3016_CN_202164315_380000_CN_24604789_380000/RConn1 -- T_24604789_380000_Schaltanlage_Ovenstädt/LConn1 -- _CN_33411203_380000_CN_24604789_380000/LConn1 -- Leitung_3018_CN_24604789_380000_CN_24230738_380000/LConn1
  Leitung_3016_CN_202164315_380000_CN_24604789_380000/RConn2 -- T_24604789_380000_Schaltanlage_Ovenstädt/LConn2 -- _CN_33411203_380000_CN_24604789_380000/LConn2 -- Leitung_3018_CN_24604789_380000_CN_24230738_380000/LConn2
  Leitung_3016_CN_202164315_380000_CN_24604789_380000/RConn3 -- T_24604789_380000_Schaltanlage_Ovenstädt/LConn3 -- _CN_33411203_380000_CN_24604789_380000/LConn3 -- Leitung_3018_CN_24604789_380000_CN_24230738_380000/LConn3
  _CN_136034396_380000_CN_28502915_380000/LConn1 -- T_136034396_380000;320000;250000_Konverterstation_Büttel/LConn1 -- _CN_136034396_380000_CN_30622610_380000/LConn1
  _CN_136034396_380000_CN_28502915_380000/LConn2 -- T_136034396_380000;320000;250000_Konverterstation_Büttel/LConn2 -- _CN_136034396_380000_CN_30622610_380000/LConn2
  _CN_136034396_380000_CN_28502915_380000/LConn3 -- T_136034396_380000;320000;250000_Konverterstation_Büttel/LConn3 -- _CN_136034396_380000_CN_30622610_380000/LConn3
  _CN_136034396_380000_CN_28502915_380000/RConn1 -- T_28502915_380000_Umspannwerk_Wilster/LConn1 -- 3105_CN_24502420_380000_CN_28502915_380000/RConn1 -- 303_CN_35176751_380000_CN_28502915_380000/LConn1
  _CN_136034396_380000_CN_28502915_380000/RConn2 -- T_28502915_380000_Umspannwerk_Wilster/LConn2 -- 3105_CN_24502420_380000_CN_28502915_380000/RConn2 -- 303_CN_35176751_380000_CN_28502915_380000/LConn2
  _CN_136034396_380000_CN_28502915_380000/RConn3 -- T_28502915_380000_Umspannwerk_Wilster/LConn3 -- 3105_CN_24502420_380000_CN_28502915_380000/RConn3 -- 303_CN_35176751_380000_CN_28502915_380000/LConn3
  _CN_136034396_380000_CN_30622610_380000/RConn1 -- T_30622610_380000;220000;110000_Umspannwerk_Kernkraftwerk_Brunsbüttel/LConn1 -- G_CN_22720647_380000_CN_30622610_380000/LConn1
  _CN_136034396_380000_CN_30622610_380000/RConn2 -- T_30622610_380000;220000;110000_Umspannwerk_Kernkraftwerk_Brunsbüttel/LConn2 -- G_CN_22720647_380000_CN_30622610_380000/LConn2
  _CN_136034396_380000_CN_30622610_380000/RConn3 -- T_30622610_380000;220000;110000_Umspannwerk_Kernkraftwerk_Brunsbüttel/LConn3 -- G_CN_22720647_380000_CN_30622610_380000/LConn3
  _CN_30164703_380000_CN58421134/LConn1 -- T_30164703_380000;110000_Graustein/LConn1 -- 565_CN_30164703_380000_CN_157806991_380000/LConn1 -- 561_CN_30164703_380000_CN_23025610_380000/LConn1
  _CN_30164703_380000_CN58421134/LConn2 -- T_30164703_380000;110000_Graustein/LConn2 -- 565_CN_30164703_380000_CN_157806991_380000/LConn2 -- 561_CN_30164703_380000_CN_23025610_380000/LConn2
  _CN_30164703_380000_CN58421134/LConn3 -- T_30164703_380000;110000_Graustein/LConn3 -- 565_CN_30164703_380000_CN_157806991_380000/LConn3 -- 561_CN_30164703_380000_CN_23025610_380000/LConn3
  G_58421134_Kraftwerk_Schwarze_Pumpe/RConn1 -- _CN_30164703_380000_CN58421134/RConn1
  G_58421134_Kraftwerk_Schwarze_Pumpe/RConn2 -- _CN_30164703_380000_CN58421134/RConn2
  G_58421134_Kraftwerk_Schwarze_Pumpe/RConn3 -- _CN_30164703_380000_CN58421134/RConn3
  565_CN_30164703_380000_CN_157806991_380000/RConn1 -- T_157806991_380000_Umspannwerk_Bärwalde/LConn1 -- 557_CN_157806991_380000_CN_157328339_380000/LConn1 -- 552_CN_157806991_380000_CN_157807291_380000/LConn1 -- MP_CN_157806991_380000_CN178167136/LConn1
  565_CN_30164703_380000_CN_157806991_380000/RConn2 -- T_157806991_380000_Umspannwerk_Bärwalde/LConn2 -- 557_CN_157806991_380000_CN_157328339_380000/LConn2 -- 552_CN_157806991_380000_CN_157807291_380000/LConn2 -- MP_CN_157806991_380000_CN178167136/LConn2
  565_CN_30164703_380000_CN_157806991_380000/RConn3 -- T_157806991_380000_Umspannwerk_Bärwalde/LConn3 -- 557_CN_157806991_380000_CN_157328339_380000/LConn3 -- 552_CN_157806991_380000_CN_157807291_380000/LConn3 -- MP_CN_157806991_380000_CN178167136/LConn3
  561_CN_30164703_380000_CN_23025610_380000/RConn1 -- T_23025610_380000;110000_Umspannwerk_Preilack/LConn1 -- 548_CN_137197826_380000_CN_23025610_380000/LConn1 -- _CN_156683994_380000_CN_23025610_380000/LConn1 -- 559_CN_157328339_380000_CN_23025610_380000/LConn1 -- _CN_23025610_380000_CN11341038/LConn1
  561_CN_30164703_380000_CN_23025610_380000/RConn2 -- T_23025610_380000;110000_Umspannwerk_Preilack/LConn2 -- 548_CN_137197826_380000_CN_23025610_380000/LConn2 -- _CN_156683994_380000_CN_23025610_380000/LConn2 -- 559_CN_157328339_380000_CN_23025610_380000/LConn2 -- _CN_23025610_380000_CN11341038/LConn2
  561_CN_30164703_380000_CN_23025610_380000/RConn3 -- T_23025610_380000;110000_Umspannwerk_Preilack/LConn3 -- 548_CN_137197826_380000_CN_23025610_380000/LConn3 -- _CN_156683994_380000_CN_23025610_380000/LConn3 -- 559_CN_157328339_380000_CN_23025610_380000/LConn3 -- _CN_23025610_380000_CN11341038/LConn3
  T_91080806_220000;110000_Umspannwerk_Pirach/LConn1 -- _CN_91080806_220000_CN167578660/LConn1
  T_91080806_220000;110000_Umspannwerk_Pirach/LConn2 -- _CN_91080806_220000_CN167578660/LConn2
  T_91080806_220000;110000_Umspannwerk_Pirach/LConn3 -- _CN_91080806_220000_CN167578660/LConn3
  _CN_91080806_220000_CN167578660/RConn1 -- G_167578660_Solarpark_Kollmann/RConn1 -- _CN_91086220_220000_CN167578660/LConn1
  _CN_91080806_220000_CN167578660/RConn2 -- G_167578660_Solarpark_Kollmann/RConn2 -- _CN_91086220_220000_CN167578660/LConn2
  _CN_91080806_220000_CN167578660/RConn3 -- G_167578660_Solarpark_Kollmann/RConn3 -- _CN_91086220_220000_CN167578660/LConn3
  T_173590639_220000;110000_Niederwiesa/LConn1 -- Röhrsdorf_CN_173590639_220000_CN_23117075_220000/LConn1
  T_173590639_220000;110000_Niederwiesa/LConn2 -- Röhrsdorf_CN_173590639_220000_CN_23117075_220000/LConn2
  T_173590639_220000;110000_Niederwiesa/LConn3 -- Röhrsdorf_CN_173590639_220000_CN_23117075_220000/LConn3
  Röhrsdorf_CN_173590639_220000_CN_23117075_220000/RConn1 -- T_23117075_380000;220000;110000_Umspannwerk_Röhrsdorf/RConn1 -- 212_Röhrsdorf___Crossen_CN_173112252_220000_CN_23117075_220000/LConn1 -- 203_Eula_CN_23117075_220000_CN_32843531_220000/LConn1 -- L_23117075/LConn1
  Röhrsdorf_CN_173590639_220000_CN_23117075_220000/RConn2 -- T_23117075_380000;220000;110000_Umspannwerk_Röhrsdorf/RConn2 -- 212_Röhrsdorf___Crossen_CN_173112252_220000_CN_23117075_220000/LConn2 -- 203_Eula_CN_23117075_220000_CN_32843531_220000/LConn2 -- L_23117075/LConn2
  Röhrsdorf_CN_173590639_220000_CN_23117075_220000/RConn3 -- T_23117075_380000;220000;110000_Umspannwerk_Röhrsdorf/RConn3 -- 212_Röhrsdorf___Crossen_CN_173112252_220000_CN_23117075_220000/LConn3 -- 203_Eula_CN_23117075_220000_CN_32843531_220000/LConn3 -- L_23117075/LConn3
  220kV_Stratum_West_CN_24479857_220000_CN_24799890_220000/LConn1 -- T_24479857_220000;110000_Station_Gellep/LConn1 -- 220kV_Stratum_West_CN_24479857_220000_CN_91854336_220000/LConn1 -- 220kV_Stratum_West_CN_24479857_220000_CN_92024105_220000/LConn1 -- 220kV_Stratum_West_CN_24479857_220000_CN_25043127_220000/LConn1
  220kV_Stratum_West_CN_24479857_220000_CN_24799890_220000/LConn2 -- T_24479857_220000;110000_Station_Gellep/LConn2 -- 220kV_Stratum_West_CN_24479857_220000_CN_91854336_220000/LConn2 -- 220kV_Stratum_West_CN_24479857_220000_CN_92024105_220000/LConn2 -- 220kV_Stratum_West_CN_24479857_220000_CN_25043127_220000/LConn2
  220kV_Stratum_West_CN_24479857_220000_CN_24799890_220000/LConn3 -- T_24479857_220000;110000_Station_Gellep/LConn3 -- 220kV_Stratum_West_CN_24479857_220000_CN_91854336_220000/LConn3 -- 220kV_Stratum_West_CN_24479857_220000_CN_92024105_220000/LConn3 -- 220kV_Stratum_West_CN_24479857_220000_CN_25043127_220000/LConn3
  220kV_Stratum_West_CN_24479857_220000_CN_24799890_220000/RConn1 -- T_24799890_220000;110000_Station_Osterath/LConn1 -- 220kV_Fichtenhain_West+Utfort_West_CN_93278553_220000_CN_24799890_220000/LConn1 -- 220kV_Neurath_1a+Osterath_West_CN_24799890_220000_CN_27919734_220000/LConn1
  220kV_Stratum_West_CN_24479857_220000_CN_24799890_220000/RConn2 -- T_24799890_220000;110000_Station_Osterath/LConn2 -- 220kV_Fichtenhain_West+Utfort_West_CN_93278553_220000_CN_24799890_220000/LConn2 -- 220kV_Neurath_1a+Osterath_West_CN_24799890_220000_CN_27919734_220000/LConn2
  220kV_Stratum_West_CN_24479857_220000_CN_24799890_220000/RConn3 -- T_24799890_220000;110000_Station_Osterath/LConn3 -- 220kV_Fichtenhain_West+Utfort_West_CN_93278553_220000_CN_24799890_220000/LConn3 -- 220kV_Neurath_1a+Osterath_West_CN_24799890_220000_CN_27919734_220000/LConn3
  220kV_Stratum_West_CN_24479857_220000_CN_91854336_220000/RConn1 -- T_91854336_220000;110000_Station_Mündelheim/LConn1 -- 220kV_Fichtenhain_West+Utfort_West_CN_93278553_220000_CN_91854336_220000/LConn1
  220kV_Stratum_West_CN_24479857_220000_CN_91854336_220000/RConn2 -- T_91854336_220000;110000_Station_Mündelheim/LConn2 -- 220kV_Fichtenhain_West+Utfort_West_CN_93278553_220000_CN_91854336_220000/LConn2
  220kV_Stratum_West_CN_24479857_220000_CN_91854336_220000/RConn3 -- T_91854336_220000;110000_Station_Mündelheim/LConn3 -- 220kV_Fichtenhain_West+Utfort_West_CN_93278553_220000_CN_91854336_220000/LConn3
  T_92024105_220000_Station_Rheinhausen/LConn1 -- 220kV_Stratum_West_CN_24479857_220000_CN_92024105_220000/RConn1
  T_92024105_220000_Station_Rheinhausen/LConn2 -- 220kV_Stratum_West_CN_24479857_220000_CN_92024105_220000/RConn2
  T_92024105_220000_Station_Rheinhausen/LConn3 -- 220kV_Stratum_West_CN_24479857_220000_CN_92024105_220000/RConn3
  T_25043127_220000;110000_Station_Selbeck/LConn1 -- 220kV_Stratum_West_CN_24479857_220000_CN_25043127_220000/RConn1
  T_25043127_220000;110000_Station_Selbeck/LConn2 -- 220kV_Stratum_West_CN_24479857_220000_CN_25043127_220000/RConn2
  T_25043127_220000;110000_Station_Selbeck/LConn3 -- 220kV_Stratum_West_CN_24479857_220000_CN_25043127_220000/RConn3
  _CN_24715381_220000_CN_276236628_220000/LConn1 -- T_24715381_380000;220000;110000_Umspannwerk_Bergrheinfeld/RConn1 -- Bergrheinfeld___Raitersaich_CN_24715381_220000_CN_24705761_220000/LConn1 -- L_24715381/LConn1
  _CN_24715381_220000_CN_276236628_220000/LConn2 -- T_24715381_380000;220000;110000_Umspannwerk_Bergrheinfeld/RConn2 -- Bergrheinfeld___Raitersaich_CN_24715381_220000_CN_24705761_220000/LConn2 -- L_24715381/LConn2
  _CN_24715381_220000_CN_276236628_220000/LConn3 -- T_24715381_380000;220000;110000_Umspannwerk_Bergrheinfeld/RConn3 -- Bergrheinfeld___Raitersaich_CN_24715381_220000_CN_24705761_220000/LConn3 -- L_24715381/LConn3
  T_276236628_220000;110000_Schweinfurt/LConn1 -- _CN_24715381_220000_CN_276236628_220000/RConn1
  T_276236628_220000;110000_Schweinfurt/LConn2 -- _CN_24715381_220000_CN_276236628_220000/RConn2
  T_276236628_220000;110000_Schweinfurt/LConn3 -- _CN_24715381_220000_CN_276236628_220000/RConn3
  Bergrheinfeld___Raitersaich_CN_24715381_220000_CN_24705761_220000/RConn1 -- T_24705761_380000;220000;110000_Umspannwerk_Raitersaich/RConn1 -- Raitersaich___Trennfeld;Trennfeld___Aschaffenburg_CN_24765111_220000_CN_24705761_220000/LConn1 -- L_24705761/LConn1
  Bergrheinfeld___Raitersaich_CN_24715381_220000_CN_24705761_220000/RConn2 -- T_24705761_380000;220000;110000_Umspannwerk_Raitersaich/RConn2 -- Raitersaich___Trennfeld;Trennfeld___Aschaffenburg_CN_24765111_220000_CN_24705761_220000/LConn2 -- L_24705761/LConn2
  Bergrheinfeld___Raitersaich_CN_24715381_220000_CN_24705761_220000/RConn3 -- T_24705761_380000;220000;110000_Umspannwerk_Raitersaich/RConn3 -- Raitersaich___Trennfeld;Trennfeld___Aschaffenburg_CN_24765111_220000_CN_24705761_220000/LConn3 -- L_24705761/LConn3
  220kV_Polsum_Süd_CN_29077623_220000_CN_23022100_220000/RConn1 -- T_23022100_380000;220000_Station_Polsum/RConn1 -- 220kV_Scholven_E_CN_23022100_220000_CN_24462426_220000/LConn1 -- 220kV_Scholven_E_CN_23022100_220000_CN22943608/LConn1 -- L_23022100/LConn1
  220kV_Polsum_Süd_CN_29077623_220000_CN_23022100_220000/RConn2 -- T_23022100_380000;220000_Station_Polsum/RConn2 -- 220kV_Scholven_E_CN_23022100_220000_CN_24462426_220000/LConn2 -- 220kV_Scholven_E_CN_23022100_220000_CN22943608/LConn2 -- L_23022100/LConn2
  220kV_Polsum_Süd_CN_29077623_220000_CN_23022100_220000/RConn3 -- T_23022100_380000;220000_Station_Polsum/RConn3 -- 220kV_Scholven_E_CN_23022100_220000_CN_24462426_220000/LConn3 -- 220kV_Scholven_E_CN_23022100_220000_CN22943608/LConn3 -- L_23022100/LConn3
  220kV_Polsum_Süd_CN_29077623_220000_CN_38584673_220000/RConn1 -- T_38584673_220000_Station_Bellendorf/LConn1 -- Scholven_C_CN_38584673_220000_CN22943608/LConn1
  220kV_Polsum_Süd_CN_29077623_220000_CN_38584673_220000/RConn2 -- T_38584673_220000_Station_Bellendorf/LConn2 -- Scholven_C_CN_38584673_220000_CN22943608/LConn2
  220kV_Polsum_Süd_CN_29077623_220000_CN_38584673_220000/RConn3 -- T_38584673_220000_Station_Bellendorf/LConn3 -- Scholven_C_CN_38584673_220000_CN22943608/LConn3
  T_22944791_220000;110000_Station_Bergmannsglück/LConn1 -- 220kV_Polsum_Süd_CN_29077623_220000_CN_22944791_220000/RConn1
  T_22944791_220000;110000_Station_Bergmannsglück/LConn2 -- 220kV_Polsum_Süd_CN_29077623_220000_CN_22944791_220000/RConn2
  T_22944791_220000;110000_Station_Bergmannsglück/LConn3 -- 220kV_Polsum_Süd_CN_29077623_220000_CN_22944791_220000/RConn3
  220kV_Polsum_Süd_CN_29077623_220000_CN_28452784_220000/RConn1 -- T_28452784_220000;110000_Station_Pöppinghausen/LConn1 -- 220kV_Cappenberg_Nord+Elmenhorst_Süd_CN_138877959_220000_CN_28452784_220000/LConn1 -- 220kV_Knepper_C_CN_28452784_220000_CN-536706/LConn1 -- _CN_66038431_220000_CN_28452784_220000/LConn1
  220kV_Polsum_Süd_CN_29077623_220000_CN_28452784_220000/RConn2 -- T_28452784_220000;110000_Station_Pöppinghausen/LConn2 -- 220kV_Cappenberg_Nord+Elmenhorst_Süd_CN_138877959_220000_CN_28452784_220000/LConn2 -- 220kV_Knepper_C_CN_28452784_220000_CN-536706/LConn2 -- _CN_66038431_220000_CN_28452784_220000/LConn2
  220kV_Polsum_Süd_CN_29077623_220000_CN_28452784_220000/RConn3 -- T_28452784_220000;110000_Station_Pöppinghausen/LConn3 -- 220kV_Cappenberg_Nord+Elmenhorst_Süd_CN_138877959_220000_CN_28452784_220000/LConn3 -- 220kV_Knepper_C_CN_28452784_220000_CN-536706/LConn3 -- _CN_66038431_220000_CN_28452784_220000/LConn3
  220kV_Polsum_Süd_CN_29077623_220000_CN_68549340_220000/RConn1 -- T_68549340_220000;110000_Station_Bochum/LConn1 -- 220kV_Welper_Ost+ANK_CN_156973363_220000_CN_68549340_220000/LConn1
  220kV_Polsum_Süd_CN_29077623_220000_CN_68549340_220000/RConn2 -- T_68549340_220000;110000_Station_Bochum/LConn2 -- 220kV_Welper_Ost+ANK_CN_156973363_220000_CN_68549340_220000/LConn2
  220kV_Polsum_Süd_CN_29077623_220000_CN_68549340_220000/RConn3 -- T_68549340_220000;110000_Station_Bochum/LConn3 -- 220kV_Welper_Ost+ANK_CN_156973363_220000_CN_68549340_220000/LConn3
  T_29282738_220000;110000_Herne/LConn1 -- 220kV_Polsum_Süd_CN_29077623_220000_CN_29282738_220000/RConn1
  T_29282738_220000;110000_Herne/LConn2 -- 220kV_Polsum_Süd_CN_29077623_220000_CN_29282738_220000/RConn2
  T_29282738_220000;110000_Herne/LConn3 -- 220kV_Polsum_Süd_CN_29077623_220000_CN_29282738_220000/RConn3
  G_25649285_Kraftwerk_Herne_Baukau/RConn1 -- 220kV_Polsum_Süd_CN_29077623_220000_CN25649285/RConn1
  G_25649285_Kraftwerk_Herne_Baukau/RConn2 -- 220kV_Polsum_Süd_CN_29077623_220000_CN25649285/RConn2
  G_25649285_Kraftwerk_Herne_Baukau/RConn3 -- 220kV_Polsum_Süd_CN_29077623_220000_CN25649285/RConn3
  _CN_29077623_380000_CN_23022100_380000/LConn1 -- T_29077623_380000;220000;110000_Station_Kusenhorst/LConn1 -- 380kV_Recklinghausen+Westfalen_West_CN_29077623_380000_CN_32472806_380000/LConn1 -- 380kV_Recklinghausen+Westfalen_West_CN_29077623_380000_CN_23067006_380000/LConn1 -- 380kV_Recklinghausen+Westfalen_West_CN_29077623_380000_CN_63114179_380000/LConn1 -- 380kV_Recklinghausen+Westfalen_West_CN_29077623_380000_CN_113546939_380000/LConn1 -- _CN_29077623_380000_CN_29471404_380000/LConn1 -- _CN_29077623_380000_CN_26383042_380000/LConn1 -- _CN_29077623_380000_CN_42560068_380000/LConn1 -- _CN_29077623_380000_CN_42488850_380000/LConn1 -- _CN_29077623_380000_CN_42507488_380000/LConn1 -- _CN_29077623_380000_CN_25506770_380000/LConn1 -- _CN_29077623_380000_CN_61918154_380000/LConn1 -- _CN_29077623_380000_CN_206289192_380000/LConn1 -- _CN_29077623_380000_CN_142487746_380000/LConn1 -- _CN_29077623_380000_CN_32042992_380000/RConn1 -- _CN_29077623_380000_CN_49299111_380000/LConn1 -- _CN_29077623_380000_CN_33411203_380000/LConn1 -- _CN_29077623_380000_CN_114319248_380000/LConn1
  _CN_29077623_380000_CN_23022100_380000/LConn2 -- T_29077623_380000;220000;110000_Station_Kusenhorst/LConn2 -- 380kV_Recklinghausen+Westfalen_West_CN_29077623_380000_CN_32472806_380000/LConn2 -- 380kV_Recklinghausen+Westfalen_West_CN_29077623_380000_CN_23067006_380000/LConn2 -- 380kV_Recklinghausen+Westfalen_West_CN_29077623_380000_CN_63114179_380000/LConn2 -- 380kV_Recklinghausen+Westfalen_West_CN_29077623_380000_CN_113546939_380000/LConn2 -- _CN_29077623_380000_CN_29471404_380000/LConn2 -- _CN_29077623_380000_CN_26383042_380000/LConn2 -- _CN_29077623_380000_CN_42560068_380000/LConn2 -- _CN_29077623_380000_CN_42488850_380000/LConn2 -- _CN_29077623_380000_CN_42507488_380000/LConn2 -- _CN_29077623_380000_CN_25506770_380000/LConn2 -- _CN_29077623_380000_CN_61918154_380000/LConn2 -- _CN_29077623_380000_CN_206289192_380000/LConn2 -- _CN_29077623_380000_CN_142487746_380000/LConn2 -- _CN_29077623_380000_CN_32042992_380000/RConn2 -- _CN_29077623_380000_CN_49299111_380000/LConn2 -- _CN_29077623_380000_CN_33411203_380000/LConn2 -- _CN_29077623_380000_CN_114319248_380000/LConn2
  _CN_29077623_380000_CN_23022100_380000/LConn3 -- T_29077623_380000;220000;110000_Station_Kusenhorst/LConn3 -- 380kV_Recklinghausen+Westfalen_West_CN_29077623_380000_CN_32472806_380000/LConn3 -- 380kV_Recklinghausen+Westfalen_West_CN_29077623_380000_CN_23067006_380000/LConn3 -- 380kV_Recklinghausen+Westfalen_West_CN_29077623_380000_CN_63114179_380000/LConn3 -- 380kV_Recklinghausen+Westfalen_West_CN_29077623_380000_CN_113546939_380000/LConn3 -- _CN_29077623_380000_CN_29471404_380000/LConn3 -- _CN_29077623_380000_CN_26383042_380000/LConn3 -- _CN_29077623_380000_CN_42560068_380000/LConn3 -- _CN_29077623_380000_CN_42488850_380000/LConn3 -- _CN_29077623_380000_CN_42507488_380000/LConn3 -- _CN_29077623_380000_CN_25506770_380000/LConn3 -- _CN_29077623_380000_CN_61918154_380000/LConn3 -- _CN_29077623_380000_CN_206289192_380000/LConn3 -- _CN_29077623_380000_CN_142487746_380000/LConn3 -- _CN_29077623_380000_CN_32042992_380000/RConn3 -- _CN_29077623_380000_CN_49299111_380000/LConn3 -- _CN_29077623_380000_CN_33411203_380000/LConn3 -- _CN_29077623_380000_CN_114319248_380000/LConn3
  _CN_29077623_380000_CN_23022100_380000/RConn1 -- T_23022100_380000;220000_Station_Polsum/LConn1 -- 380kV_Lippe_Süd_CN_23022100_380000_CN_24462426_380000/LConn1 -- 380kV_Kusenhorst_CN_23022100_380000_CN_24280460_380000/LConn1 -- 380kV_Kusenhorst_CN_23022100_380000_CN_26291794_380000/LConn1 -- 380kV_Kusenhorst_CN_23022100_380000_CN_24921206_380000/LConn1 -- 380kV_Scholven_B_CN_23022100_380000_CN22943608/LConn1
  _CN_29077623_380000_CN_23022100_380000/RConn2 -- T_23022100_380000;220000_Station_Polsum/LConn2 -- 380kV_Lippe_Süd_CN_23022100_380000_CN_24462426_380000/LConn2 -- 380kV_Kusenhorst_CN_23022100_380000_CN_24280460_380000/LConn2 -- 380kV_Kusenhorst_CN_23022100_380000_CN_26291794_380000/LConn2 -- 380kV_Kusenhorst_CN_23022100_380000_CN_24921206_380000/LConn2 -- 380kV_Scholven_B_CN_23022100_380000_CN22943608/LConn2
  _CN_29077623_380000_CN_23022100_380000/RConn3 -- T_23022100_380000;220000_Station_Polsum/LConn3 -- 380kV_Lippe_Süd_CN_23022100_380000_CN_24462426_380000/LConn3 -- 380kV_Kusenhorst_CN_23022100_380000_CN_24280460_380000/LConn3 -- 380kV_Kusenhorst_CN_23022100_380000_CN_26291794_380000/LConn3 -- 380kV_Kusenhorst_CN_23022100_380000_CN_24921206_380000/LConn3 -- 380kV_Scholven_B_CN_23022100_380000_CN22943608/LConn3
  380kV_Recklinghausen+Westfalen_West_CN_29077623_380000_CN_32472806_380000/RConn1 -- T_32472806_380000_Station_Mengede/LConn1 -- _CN_42488855_380000_CN_32472806_380000/LConn1 -- 380kV_Mengede_Nord+Süd_CN_121199242_380000_CN_32472806_380000/LConn1
  380kV_Recklinghausen+Westfalen_West_CN_29077623_380000_CN_32472806_380000/RConn2 -- T_32472806_380000_Station_Mengede/LConn2 -- _CN_42488855_380000_CN_32472806_380000/LConn2 -- 380kV_Mengede_Nord+Süd_CN_121199242_380000_CN_32472806_380000/LConn2
  380kV_Recklinghausen+Westfalen_West_CN_29077623_380000_CN_32472806_380000/RConn3 -- T_32472806_380000_Station_Mengede/LConn3 -- _CN_42488855_380000_CN_32472806_380000/LConn3 -- 380kV_Mengede_Nord+Süd_CN_121199242_380000_CN_32472806_380000/LConn3
  T_23067006_380000;110000_Station_Hüllen/LConn1 -- 380kV_Recklinghausen+Westfalen_West_CN_29077623_380000_CN_23067006_380000/RConn1
  T_23067006_380000;110000_Station_Hüllen/LConn2 -- 380kV_Recklinghausen+Westfalen_West_CN_29077623_380000_CN_23067006_380000/RConn2
  T_23067006_380000;110000_Station_Hüllen/LConn3 -- 380kV_Recklinghausen+Westfalen_West_CN_29077623_380000_CN_23067006_380000/RConn3
  380kV_Recklinghausen+Westfalen_West_CN_29077623_380000_CN_63114179_380000/RConn1 -- T_63114179_380000;220000;110000_Station_Hattingen/LConn1 -- _CN_63114179_380000_CN_35763480_380000/LConn1
  380kV_Recklinghausen+Westfalen_West_CN_29077623_380000_CN_63114179_380000/RConn2 -- T_63114179_380000;220000;110000_Station_Hattingen/LConn2 -- _CN_63114179_380000_CN_35763480_380000/LConn2
  380kV_Recklinghausen+Westfalen_West_CN_29077623_380000_CN_63114179_380000/RConn3 -- T_63114179_380000;220000;110000_Station_Hattingen/LConn3 -- _CN_63114179_380000_CN_35763480_380000/LConn3
  380kV_Recklinghausen+Westfalen_West_CN_29077623_380000_CN_113546939_380000/RConn1 -- T_113546939_380000;220000_Station_Eiberg/LConn1 -- 380_kV_Neurath_2b;_Oerkhaus_Ost_CN_22761839_380000_CN_113546939_380000/LConn1 -- _CN_59925390_380000_CN_113546939_380000/LConn1
  380kV_Recklinghausen+Westfalen_West_CN_29077623_380000_CN_113546939_380000/RConn2 -- T_113546939_380000;220000_Station_Eiberg/LConn2 -- 380_kV_Neurath_2b;_Oerkhaus_Ost_CN_22761839_380000_CN_113546939_380000/LConn2 -- _CN_59925390_380000_CN_113546939_380000/LConn2
  380kV_Recklinghausen+Westfalen_West_CN_29077623_380000_CN_113546939_380000/RConn3 -- T_113546939_380000;220000_Station_Eiberg/LConn3 -- 380_kV_Neurath_2b;_Oerkhaus_Ost_CN_22761839_380000_CN_113546939_380000/LConn3 -- _CN_59925390_380000_CN_113546939_380000/LConn3
  T_29471404_380000;220000;110000_Station_Gronau/LConn1 -- _CN_29077623_380000_CN_29471404_380000/RConn1
  T_29471404_380000;220000;110000_Station_Gronau/LConn2 -- _CN_29077623_380000_CN_29471404_380000/RConn2
  T_29471404_380000;220000;110000_Station_Gronau/LConn3 -- _CN_29077623_380000_CN_29471404_380000/RConn3
  _CN_29077623_380000_CN_26383042_380000/RConn1 -- T_26383042_380000;220000;110000;10000_Umspannwerk_Blankenhagen/LConn1 -- _CN_26383042_380000_CN_24264701_380000/LConn1
  _CN_29077623_380000_CN_26383042_380000/RConn2 -- T_26383042_380000;220000;110000;10000_Umspannwerk_Blankenhagen/LConn2 -- _CN_26383042_380000_CN_24264701_380000/LConn2
  _CN_29077623_380000_CN_26383042_380000/RConn3 -- T_26383042_380000;220000;110000;10000_Umspannwerk_Blankenhagen/LConn3 -- _CN_26383042_380000_CN_24264701_380000/LConn3
  T_42560068_380000;110000_Station_Enniger/LConn1 -- _CN_29077623_380000_CN_42560068_380000/RConn1
  T_42560068_380000;110000_Station_Enniger/LConn2 -- _CN_29077623_380000_CN_42560068_380000/RConn2
  T_42560068_380000;110000_Station_Enniger/LConn3 -- _CN_29077623_380000_CN_42560068_380000/RConn3
  _CN_29077623_380000_CN_42488850_380000/RConn1 -- T_42488850_380000_Station_Uentrop/LConn1 -- _CN_42488855_380000_CN_42488850_380000/LConn1 -- 380kV_Sauerland_Süd_CN_42799487_380000_CN_42488850_380000/LConn1 -- 380kV_Westfalen_D+E_CN_202580524_380000_CN_42488850_380000/LConn1
  _CN_29077623_380000_CN_42488850_380000/RConn2 -- T_42488850_380000_Station_Uentrop/LConn2 -- _CN_42488855_380000_CN_42488850_380000/LConn2 -- 380kV_Sauerland_Süd_CN_42799487_380000_CN_42488850_380000/LConn2 -- 380kV_Westfalen_D+E_CN_202580524_380000_CN_42488850_380000/LConn2
  _CN_29077623_380000_CN_42488850_380000/RConn3 -- T_42488850_380000_Station_Uentrop/LConn3 -- _CN_42488855_380000_CN_42488850_380000/LConn3 -- 380kV_Sauerland_Süd_CN_42799487_380000_CN_42488850_380000/LConn3 -- 380kV_Westfalen_D+E_CN_202580524_380000_CN_42488850_380000/LConn3
  _CN_29077623_380000_CN_42507488_380000/RConn1 -- T_42507488_380000;220000;110000_Station_Gersteinwerk/LConn1 -- 380kV_Waltrop_Süd_CN_121199242_380000_CN_42507488_380000/LConn1 -- 380kV_Gersteinwerk_K2_CN_42507488_380000_CN33883956/LConn1
  _CN_29077623_380000_CN_42507488_380000/RConn2 -- T_42507488_380000;220000;110000_Station_Gersteinwerk/LConn2 -- 380kV_Waltrop_Süd_CN_121199242_380000_CN_42507488_380000/LConn2 -- 380kV_Gersteinwerk_K2_CN_42507488_380000_CN33883956/LConn2
  _CN_29077623_380000_CN_42507488_380000/RConn3 -- T_42507488_380000;220000;110000_Station_Gersteinwerk/LConn3 -- 380kV_Waltrop_Süd_CN_121199242_380000_CN_42507488_380000/LConn3 -- 380kV_Gersteinwerk_K2_CN_42507488_380000_CN33883956/LConn3
  T_25506770_380000;110000_Station_Roxel/LConn1 -- _CN_29077623_380000_CN_25506770_380000/RConn1
  T_25506770_380000;110000_Station_Roxel/LConn2 -- _CN_29077623_380000_CN_25506770_380000/RConn2
  T_25506770_380000;110000_Station_Roxel/LConn3 -- _CN_29077623_380000_CN_25506770_380000/RConn3
  _CN_29077623_380000_CN_61918154_380000/RConn1 -- T_61918154_380000;220000;110000_Hanekenfähr/LConn1 -- 380_kV_Kernkraftwerk_Emsland_CN_61918154_380000_CN43912398/LConn1 -- _CN_61918154_380000_CN49339874/LConn1
  _CN_29077623_380000_CN_61918154_380000/RConn2 -- T_61918154_380000;220000;110000_Hanekenfähr/LConn2 -- 380_kV_Kernkraftwerk_Emsland_CN_61918154_380000_CN43912398/LConn2 -- _CN_61918154_380000_CN49339874/LConn2
  _CN_29077623_380000_CN_61918154_380000/RConn3 -- T_61918154_380000;220000;110000_Hanekenfähr/LConn3 -- 380_kV_Kernkraftwerk_Emsland_CN_61918154_380000_CN43912398/LConn3 -- _CN_61918154_380000_CN49339874/LConn3
  T_206289192_380000;110000_Meppen/LConn1 -- _CN_29077623_380000_CN_206289192_380000/RConn1
  T_206289192_380000;110000_Meppen/LConn2 -- _CN_29077623_380000_CN_206289192_380000/RConn2
  T_206289192_380000;110000_Meppen/LConn3 -- _CN_29077623_380000_CN_206289192_380000/RConn3
  T_142487746_380000;320000_Dörpen_West/LConn1 -- _CN_29077623_380000_CN_142487746_380000/RConn1
  T_142487746_380000;320000_Dörpen_West/LConn2 -- _CN_29077623_380000_CN_142487746_380000/RConn2
  T_142487746_380000;320000_Dörpen_West/LConn3 -- _CN_29077623_380000_CN_142487746_380000/RConn3
  T_49299111_380000;110000_Niederlangen/LConn1 -- _CN_29077623_380000_CN_49299111_380000/RConn1
  T_49299111_380000;110000_Niederlangen/LConn2 -- _CN_29077623_380000_CN_49299111_380000/RConn2
  T_49299111_380000;110000_Niederlangen/LConn3 -- _CN_29077623_380000_CN_49299111_380000/RConn3
  _CN_29077623_380000_CN_33411203_380000/RConn1 -- T_33411203_380000;220000;110000_Wehrendorf/LConn1 -- _CN_33411203_380000_CN_27739871_380000/RConn1 -- _CN_33411203_380000_CN_24604789_380000/RConn1
  _CN_29077623_380000_CN_33411203_380000/RConn2 -- T_33411203_380000;220000;110000_Wehrendorf/LConn2 -- _CN_33411203_380000_CN_27739871_380000/RConn2 -- _CN_33411203_380000_CN_24604789_380000/RConn2
  _CN_29077623_380000_CN_33411203_380000/RConn3 -- T_33411203_380000;220000;110000_Wehrendorf/LConn3 -- _CN_33411203_380000_CN_27739871_380000/RConn3 -- _CN_33411203_380000_CN_24604789_380000/RConn3
  T_114319248_380000;220000;110000_Station_Westerkappeln/LConn1 -- _CN_29077623_380000_CN_114319248_380000/RConn1
  T_114319248_380000;220000;110000_Station_Westerkappeln/LConn2 -- _CN_29077623_380000_CN_114319248_380000/RConn2
  T_114319248_380000;220000;110000_Station_Westerkappeln/LConn3 -- _CN_29077623_380000_CN_114319248_380000/RConn3
  T_39690368_220000;110000_Güstrow/LConn1 -- _CN_39690368_220000_CN_32062544_220000/LConn1
  T_39690368_220000;110000_Güstrow/LConn2 -- _CN_39690368_220000_CN_32062544_220000/LConn2
  T_39690368_220000;110000_Güstrow/LConn3 -- _CN_39690368_220000_CN_32062544_220000/LConn3
  _CN_39690368_220000_CN_32062544_220000/RConn1 -- T_32062544_380000;220000_Güstrow/RConn1 -- _CN_32318130_220000_CN_32062544_220000/LConn1 -- L_32062544/LConn1
  _CN_39690368_220000_CN_32062544_220000/RConn2 -- T_32062544_380000;220000_Güstrow/RConn2 -- _CN_32318130_220000_CN_32062544_220000/LConn2 -- L_32062544/LConn2
  _CN_39690368_220000_CN_32062544_220000/RConn3 -- T_32062544_380000;220000_Güstrow/RConn3 -- _CN_32318130_220000_CN_32062544_220000/LConn3 -- L_32062544/LConn3
  _CN_33411203_220000_CN_37764852_220000/RConn1 -- T_33411203_380000;220000;110000_Wehrendorf/RConn1 -- _CN_33411203_220000_CN_114319248_220000/RConn1 -- 220kV_Diepholz_Ost_CN_33411203_220000_CN_32904794_220000/LConn1 -- L_33411203/LConn1
  _CN_33411203_220000_CN_37764852_220000/RConn2 -- T_33411203_380000;220000;110000_Wehrendorf/RConn2 -- _CN_33411203_220000_CN_114319248_220000/RConn2 -- 220kV_Diepholz_Ost_CN_33411203_220000_CN_32904794_220000/LConn2 -- L_33411203/LConn2
  _CN_33411203_220000_CN_37764852_220000/RConn3 -- T_33411203_380000;220000;110000_Wehrendorf/RConn3 -- _CN_33411203_220000_CN_114319248_220000/RConn3 -- 220kV_Diepholz_Ost_CN_33411203_220000_CN_32904794_220000/LConn3 -- L_33411203/LConn3
  T_32904794_220000;110000_Station_Sankt_Hülfe/LConn1 -- 220kV_Diepholz_Ost_CN_33411203_220000_CN_32904794_220000/RConn1
  T_32904794_220000;110000_Station_Sankt_Hülfe/LConn2 -- 220kV_Diepholz_Ost_CN_33411203_220000_CN_32904794_220000/RConn2
  T_32904794_220000;110000_Station_Sankt_Hülfe/LConn3 -- 220kV_Diepholz_Ost_CN_33411203_220000_CN_32904794_220000/RConn3
  _CN_22720647_220000_CN_28008024_220000/RConn1 -- T_22720647_380000;220000;110000_Umspannwerk_Hamburg_Nord/RConn1 -- L_22720647/LConn1
  _CN_22720647_220000_CN_28008024_220000/RConn2 -- T_22720647_380000;220000;110000_Umspannwerk_Hamburg_Nord/RConn2 -- L_22720647/LConn2
  _CN_22720647_220000_CN_28008024_220000/RConn3 -- T_22720647_380000;220000;110000_Umspannwerk_Hamburg_Nord/RConn3 -- L_22720647/LConn3
  G_CN_22720647_380000_CN_30622610_380000/RConn1 -- T_22720647_380000;220000;110000_Umspannwerk_Hamburg_Nord/LConn1 -- _CN_22720647_380000_CN_23583867_380000/LConn1
  G_CN_22720647_380000_CN_30622610_380000/RConn2 -- T_22720647_380000;220000;110000_Umspannwerk_Hamburg_Nord/LConn2 -- _CN_22720647_380000_CN_23583867_380000/LConn2
  G_CN_22720647_380000_CN_30622610_380000/RConn3 -- T_22720647_380000;220000;110000_Umspannwerk_Hamburg_Nord/LConn3 -- _CN_22720647_380000_CN_23583867_380000/LConn3
  _CN_22720647_380000_CN_23583867_380000/RConn1 -- T_23583867_380000;110000_Umspannwerk_Hamburg_Ost/LConn1 -- KKW_Krümmel___UW_HH_OST_CN_23366603_380000_CN_23583867_380000/LConn1 -- D_CN_23583867_380000_CN_11285720_380000/LConn1
  _CN_22720647_380000_CN_23583867_380000/RConn2 -- T_23583867_380000;110000_Umspannwerk_Hamburg_Ost/LConn2 -- KKW_Krümmel___UW_HH_OST_CN_23366603_380000_CN_23583867_380000/LConn2 -- D_CN_23583867_380000_CN_11285720_380000/LConn2
  _CN_22720647_380000_CN_23583867_380000/RConn3 -- T_23583867_380000;110000_Umspannwerk_Hamburg_Ost/LConn3 -- KKW_Krümmel___UW_HH_OST_CN_23366603_380000_CN_23583867_380000/LConn3 -- D_CN_23583867_380000_CN_11285720_380000/LConn3
  _CN_42488855_380000_CN_112695048_380000/LConn1 -- T_42488855_380000;110000_Station_Lippborg/LConn1 -- _CN_42488855_380000_CN_42809973_380000/LConn1 -- _CN_42488855_380000_CN_35763480_380000/LConn1 -- _CN_42488855_380000_CN_22964137_380000/LConn1 -- _CN_42488855_380000_CN_32472806_380000/RConn1 -- _CN_42488855_380000_CN_42488850_380000/RConn1
  _CN_42488855_380000_CN_112695048_380000/LConn2 -- T_42488855_380000;110000_Station_Lippborg/LConn2 -- _CN_42488855_380000_CN_42809973_380000/LConn2 -- _CN_42488855_380000_CN_35763480_380000/LConn2 -- _CN_42488855_380000_CN_22964137_380000/LConn2 -- _CN_42488855_380000_CN_32472806_380000/RConn2 -- _CN_42488855_380000_CN_42488850_380000/RConn2
  _CN_42488855_380000_CN_112695048_380000/LConn3 -- T_42488855_380000;110000_Station_Lippborg/LConn3 -- _CN_42488855_380000_CN_42809973_380000/LConn3 -- _CN_42488855_380000_CN_35763480_380000/LConn3 -- _CN_42488855_380000_CN_22964137_380000/LConn3 -- _CN_42488855_380000_CN_32472806_380000/RConn3 -- _CN_42488855_380000_CN_42488850_380000/RConn3
  T_112695048_380000_Geithe/LConn1 -- _CN_42488855_380000_CN_112695048_380000/RConn1
  T_112695048_380000_Geithe/LConn2 -- _CN_42488855_380000_CN_112695048_380000/RConn2
  T_112695048_380000_Geithe/LConn3 -- _CN_42488855_380000_CN_112695048_380000/RConn3
  T_42809973_380000;110000_Station_Unna/LConn1 -- _CN_42488855_380000_CN_42809973_380000/RConn1
  T_42809973_380000;110000_Station_Unna/LConn2 -- _CN_42488855_380000_CN_42809973_380000/RConn2
  T_42809973_380000;110000_Station_Unna/LConn3 -- _CN_42488855_380000_CN_42809973_380000/RConn3
  _CN_42488855_380000_CN_35763480_380000/RConn1 -- T_35763480_380000_Witten/LConn1 -- Trafo_411_CN_35763480_380000_CN_35763481_380000/LConn1 -- _CN_63114179_380000_CN_35763480_380000/RConn1
  _CN_42488855_380000_CN_35763480_380000/RConn2 -- T_35763480_380000_Witten/LConn2 -- Trafo_411_CN_35763480_380000_CN_35763481_380000/LConn2 -- _CN_63114179_380000_CN_35763480_380000/RConn2
  _CN_42488855_380000_CN_35763480_380000/RConn3 -- T_35763480_380000_Witten/LConn3 -- Trafo_411_CN_35763480_380000_CN_35763481_380000/LConn3 -- _CN_63114179_380000_CN_35763480_380000/RConn3
  T_22964137_380000;220000;110000_Station_Kruckel/LConn1 -- _CN_42488855_380000_CN_22964137_380000/RConn1
  T_22964137_380000;220000;110000_Station_Kruckel/LConn2 -- _CN_42488855_380000_CN_22964137_380000/RConn2
  T_22964137_380000;220000;110000_Station_Kruckel/LConn3 -- _CN_42488855_380000_CN_22964137_380000/RConn3
  514_CN_59707532_380000_CN_33169401_380000/LConn1 -- T_59707532_380000;110000_Umspannwerk_Perleberg/LConn1 -- 514_CN_59707532_380000_CN_32062544_380000/RConn1 -- 514_CN_59707532_380000_CN_29877599_380000/LConn1 -- 514_CN_59707532_380000_CN_369680693_380000/LConn1
  514_CN_59707532_380000_CN_33169401_380000/LConn2 -- T_59707532_380000;110000_Umspannwerk_Perleberg/LConn2 -- 514_CN_59707532_380000_CN_32062544_380000/RConn2 -- 514_CN_59707532_380000_CN_29877599_380000/LConn2 -- 514_CN_59707532_380000_CN_369680693_380000/LConn2
  514_CN_59707532_380000_CN_33169401_380000/LConn3 -- T_59707532_380000;110000_Umspannwerk_Perleberg/LConn3 -- 514_CN_59707532_380000_CN_32062544_380000/RConn3 -- 514_CN_59707532_380000_CN_29877599_380000/LConn3 -- 514_CN_59707532_380000_CN_369680693_380000/LConn3
  514_CN_59707532_380000_CN_33169401_380000/RConn1 -- T_33169401_380000;110000_Stendal_West/LConn1 -- 490_CN_26472665_380000_CN_33169401_380000/LConn1
  514_CN_59707532_380000_CN_33169401_380000/RConn2 -- T_33169401_380000;110000_Stendal_West/LConn2 -- 490_CN_26472665_380000_CN_33169401_380000/LConn2
  514_CN_59707532_380000_CN_33169401_380000/RConn3 -- T_33169401_380000;110000_Stendal_West/LConn3 -- 490_CN_26472665_380000_CN_33169401_380000/LConn3
  514_CN_59707532_380000_CN_29877599_380000/RConn1 -- T_29877599_380000;220000_Umspannwerk_Lubmin/LConn1 -- 517_CN_137197826_380000_CN_29877599_380000/LConn1
  514_CN_59707532_380000_CN_29877599_380000/RConn2 -- T_29877599_380000;220000_Umspannwerk_Lubmin/LConn2 -- 517_CN_137197826_380000_CN_29877599_380000/LConn2
  514_CN_59707532_380000_CN_29877599_380000/RConn3 -- T_29877599_380000;220000_Umspannwerk_Lubmin/LConn3 -- 517_CN_137197826_380000_CN_29877599_380000/LConn3
  T_369680693_380000;110000_Siedenbrünzow/LConn1 -- 514_CN_59707532_380000_CN_369680693_380000/RConn1
  T_369680693_380000;110000_Siedenbrünzow/LConn2 -- 514_CN_59707532_380000_CN_369680693_380000/RConn2
  T_369680693_380000;110000_Siedenbrünzow/LConn3 -- 514_CN_59707532_380000_CN_369680693_380000/RConn3
  220_kV_Kondelwald;_220kV_Wengerohr_CN_66764943_220000_CN_145680894_220000/LConn1 -- T_66764943_220000;110000_Station_Wengerohr/LConn1 -- 220_kV_Kondelwald;_220kV_Wengerohr_CN_66764943_220000_CN_151967291_220000/LConn1 -- 220_kV_Kondelwald;_220kV_Wengerohr_CN_66764943_220000_CN_54359256_220000/LConn1 -- 220_kV_Kondelwald;_220kV_Wengerohr_CN_66764943_220000_CN28051874/LConn1 -- 220_kV_Kondelwald;_220kV_Wengerohr_CN_66764943_220000_CN_156402422_220000/LConn1 -- 220_kV_Kondelwald;_220kV_Wengerohr_CN_66764943_220000_CN_152107810_220000/LConn1 -- 220_kV_Kondelwald;_220kV_Wengerohr_CN_66764943_220000_CN_276249131_220000/LConn1 -- 220_kV_Kondelwald;_220kV_Wengerohr_CN_66764943_220000_CN_152261133_220000/RConn1 -- 220_kV_Kondelwald;_220kV_Wengerohr_CN_66764943_220000_CN_152924498_220000/LConn1 -- 220_kV_Kondelwald;_220kV_Wengerohr_CN_66764943_220000_CN_152924508_220000/LConn1 -- 220_kV_Kondelwald;_220kV_Wengerohr_CN_66764943_220000_CN_149987048_220000/RConn1 -- 220_kV_Kondelwald;_220kV_Wengerohr_CN_66764943_220000_CN_152107815_220000/LConn1 -- 220_kV_Kondelwald;_220kV_Wengerohr_CN_66764943_220000_CN_151967290_220000/LConn1 -- 220_kV_Kondelwald;_220kV_Wengerohr_CN_66764943_220000_CN_395847307_220000/LConn1
  220_kV_Kondelwald;_220kV_Wengerohr_CN_66764943_220000_CN_145680894_220000/LConn2 -- T_66764943_220000;110000_Station_Wengerohr/LConn2 -- 220_kV_Kondelwald;_220kV_Wengerohr_CN_66764943_220000_CN_151967291_220000/LConn2 -- 220_kV_Kondelwald;_220kV_Wengerohr_CN_66764943_220000_CN_54359256_220000/LConn2 -- 220_kV_Kondelwald;_220kV_Wengerohr_CN_66764943_220000_CN28051874/LConn2 -- 220_kV_Kondelwald;_220kV_Wengerohr_CN_66764943_220000_CN_156402422_220000/LConn2 -- 220_kV_Kondelwald;_220kV_Wengerohr_CN_66764943_220000_CN_152107810_220000/LConn2 -- 220_kV_Kondelwald;_220kV_Wengerohr_CN_66764943_220000_CN_276249131_220000/LConn2 -- 220_kV_Kondelwald;_220kV_Wengerohr_CN_66764943_220000_CN_152261133_220000/RConn2 -- 220_kV_Kondelwald;_220kV_Wengerohr_CN_66764943_220000_CN_152924498_220000/LConn2 -- 220_kV_Kondelwald;_220kV_Wengerohr_CN_66764943_220000_CN_152924508_220000/LConn2 -- 220_kV_Kondelwald;_220kV_Wengerohr_CN_66764943_220000_CN_149987048_220000/RConn2 -- 220_kV_Kondelwald;_220kV_Wengerohr_CN_66764943_220000_CN_152107815_220000/LConn2 -- 220_kV_Kondelwald;_220kV_Wengerohr_CN_66764943_220000_CN_151967290_220000/LConn2 -- 220_kV_Kondelwald;_220kV_Wengerohr_CN_66764943_220000_CN_395847307_220000/LConn2
  220_kV_Kondelwald;_220kV_Wengerohr_CN_66764943_220000_CN_145680894_220000/LConn3 -- T_66764943_220000;110000_Station_Wengerohr/LConn3 -- 220_kV_Kondelwald;_220kV_Wengerohr_CN_66764943_220000_CN_151967291_220000/LConn3 -- 220_kV_Kondelwald;_220kV_Wengerohr_CN_66764943_220000_CN_54359256_220000/LConn3 -- 220_kV_Kondelwald;_220kV_Wengerohr_CN_66764943_220000_CN28051874/LConn3 -- 220_kV_Kondelwald;_220kV_Wengerohr_CN_66764943_220000_CN_156402422_220000/LConn3 -- 220_kV_Kondelwald;_220kV_Wengerohr_CN_66764943_220000_CN_152107810_220000/LConn3 -- 220_kV_Kondelwald;_220kV_Wengerohr_CN_66764943_220000_CN_276249131_220000/LConn3 -- 220_kV_Kondelwald;_220kV_Wengerohr_CN_66764943_220000_CN_152261133_220000/RConn3 -- 220_kV_Kondelwald;_220kV_Wengerohr_CN_66764943_220000_CN_152924498_220000/LConn3 -- 220_kV_Kondelwald;_220kV_Wengerohr_CN_66764943_220000_CN_152924508_220000/LConn3 -- 220_kV_Kondelwald;_220kV_Wengerohr_CN_66764943_220000_CN_149987048_220000/RConn3 -- 220_kV_Kondelwald;_220kV_Wengerohr_CN_66764943_220000_CN_152107815_220000/LConn3 -- 220_kV_Kondelwald;_220kV_Wengerohr_CN_66764943_220000_CN_151967290_220000/LConn3 -- 220_kV_Kondelwald;_220kV_Wengerohr_CN_66764943_220000_CN_395847307_220000/LConn3
  220_kV_Kondelwald;_220kV_Wengerohr_CN_66764943_220000_CN_145680894_220000/RConn1 -- T_145680894_220000_Station_Trier/LConn1 -- _CN_89215122_220000_CN_145680894_220000/LConn1
  220_kV_Kondelwald;_220kV_Wengerohr_CN_66764943_220000_CN_145680894_220000/RConn2 -- T_145680894_220000_Station_Trier/LConn2 -- _CN_89215122_220000_CN_145680894_220000/LConn2
  220_kV_Kondelwald;_220kV_Wengerohr_CN_66764943_220000_CN_145680894_220000/RConn3 -- T_145680894_220000_Station_Trier/LConn3 -- _CN_89215122_220000_CN_145680894_220000/LConn3
  T_151967291_220000;110000_Station_Quint/LConn1 -- 220_kV_Kondelwald;_220kV_Wengerohr_CN_66764943_220000_CN_151967291_220000/RConn1
  T_151967291_220000;110000_Station_Quint/LConn2 -- 220_kV_Kondelwald;_220kV_Wengerohr_CN_66764943_220000_CN_151967291_220000/RConn2
  T_151967291_220000;110000_Station_Quint/LConn3 -- 220_kV_Kondelwald;_220kV_Wengerohr_CN_66764943_220000_CN_151967291_220000/RConn3
  220_kV_Kondelwald;_220kV_Wengerohr_CN_66764943_220000_CN_54359256_220000/RConn1 -- T_54359256_380000;220000;110000_Umspannwerk_Uchtelfangen/RConn1 -- _CN_89215122_220000_CN_54359256_220000/LConn1 -- _CN_54359256_220000_CN_100812630_220000/LConn1 -- _CN_54359256_220000_CN30425117/LConn1 -- L_54359256/LConn1
  220_kV_Kondelwald;_220kV_Wengerohr_CN_66764943_220000_CN_54359256_220000/RConn2 -- T_54359256_380000;220000;110000_Umspannwerk_Uchtelfangen/RConn2 -- _CN_89215122_220000_CN_54359256_220000/LConn2 -- _CN_54359256_220000_CN_100812630_220000/LConn2 -- _CN_54359256_220000_CN30425117/LConn2 -- L_54359256/LConn2
  220_kV_Kondelwald;_220kV_Wengerohr_CN_66764943_220000_CN_54359256_220000/RConn3 -- T_54359256_380000;220000;110000_Umspannwerk_Uchtelfangen/RConn3 -- _CN_89215122_220000_CN_54359256_220000/LConn3 -- _CN_54359256_220000_CN_100812630_220000/LConn3 -- _CN_54359256_220000_CN30425117/LConn3 -- L_54359256/LConn3
  220_kV_Kondelwald;_220kV_Wengerohr_CN_66764943_220000_CN28051874/RConn1 -- G_28051874_Kraftwerk_Bexbach/RConn1 -- _CN_89352550_380000_CN28051874/LConn1 -- _CN_89352550_220000_CN28051874/LConn1 -- _CN_152018146_380000_CN28051874/LConn1
  220_kV_Kondelwald;_220kV_Wengerohr_CN_66764943_220000_CN28051874/RConn2 -- G_28051874_Kraftwerk_Bexbach/RConn2 -- _CN_89352550_380000_CN28051874/LConn2 -- _CN_89352550_220000_CN28051874/LConn2 -- _CN_152018146_380000_CN28051874/LConn2
  220_kV_Kondelwald;_220kV_Wengerohr_CN_66764943_220000_CN28051874/RConn3 -- G_28051874_Kraftwerk_Bexbach/RConn3 -- _CN_89352550_380000_CN28051874/LConn3 -- _CN_89352550_220000_CN28051874/LConn3 -- _CN_152018146_380000_CN28051874/LConn3
  T_156402422_220000;110000_Beeden/LConn1 -- 220_kV_Kondelwald;_220kV_Wengerohr_CN_66764943_220000_CN_156402422_220000/RConn1
  T_156402422_220000;110000_Beeden/LConn2 -- 220_kV_Kondelwald;_220kV_Wengerohr_CN_66764943_220000_CN_156402422_220000/RConn2
  T_156402422_220000;110000_Beeden/LConn3 -- 220_kV_Kondelwald;_220kV_Wengerohr_CN_66764943_220000_CN_156402422_220000/RConn3
  T_152107810_220000;110000_Umspannwerk_Kerzenheim/LConn1 -- 220_kV_Kondelwald;_220kV_Wengerohr_CN_66764943_220000_CN_152107810_220000/RConn1
  T_152107810_220000;110000_Umspannwerk_Kerzenheim/LConn2 -- 220_kV_Kondelwald;_220kV_Wengerohr_CN_66764943_220000_CN_152107810_220000/RConn2
  T_152107810_220000;110000_Umspannwerk_Kerzenheim/LConn3 -- 220_kV_Kondelwald;_220kV_Wengerohr_CN_66764943_220000_CN_152107810_220000/RConn3
  T_276249131_220000;110000_Umspannwerk_Maximiliansau/LConn1 -- 220_kV_Kondelwald;_220kV_Wengerohr_CN_66764943_220000_CN_276249131_220000/RConn1
  T_276249131_220000;110000_Umspannwerk_Maximiliansau/LConn2 -- 220_kV_Kondelwald;_220kV_Wengerohr_CN_66764943_220000_CN_276249131_220000/RConn2
  T_276249131_220000;110000_Umspannwerk_Maximiliansau/LConn3 -- 220_kV_Kondelwald;_220kV_Wengerohr_CN_66764943_220000_CN_276249131_220000/RConn3
  220_kV_Kondelwald;_220kV_Wengerohr_CN_66764943_220000_CN_152924498_220000/RConn1 -- T_152924498_220000;110000_Netzleitstelle_Mutterstadt/LConn1 -- _CN_152924498_220000_CN152506744/LConn1
  220_kV_Kondelwald;_220kV_Wengerohr_CN_66764943_220000_CN_152924498_220000/RConn2 -- T_152924498_220000;110000_Netzleitstelle_Mutterstadt/LConn2 -- _CN_152924498_220000_CN152506744/LConn2
  220_kV_Kondelwald;_220kV_Wengerohr_CN_66764943_220000_CN_152924498_220000/RConn3 -- T_152924498_220000;110000_Netzleitstelle_Mutterstadt/LConn3 -- _CN_152924498_220000_CN152506744/LConn3
  220_kV_Kondelwald;_220kV_Wengerohr_CN_66764943_220000_CN_152924508_220000/RConn1 -- T_152924508_220000_BASF/LConn1 -- 220_kV_Anilin_1A|2B_CN_152924508_220000_CN_149987048_220000/RConn1
  220_kV_Kondelwald;_220kV_Wengerohr_CN_66764943_220000_CN_152924508_220000/RConn2 -- T_152924508_220000_BASF/LConn2 -- 220_kV_Anilin_1A|2B_CN_152924508_220000_CN_149987048_220000/RConn2
  220_kV_Kondelwald;_220kV_Wengerohr_CN_66764943_220000_CN_152924508_220000/RConn3 -- T_152924508_220000_BASF/LConn3 -- 220_kV_Anilin_1A|2B_CN_152924508_220000_CN_149987048_220000/RConn3
  220_kV_Kondelwald;_220kV_Wengerohr_CN_66764943_220000_CN_152107815_220000/RConn1 -- T_152107815_220000;110000_Otterbach/LConn1 -- _CN_152107815_220000_CN_152022992_220000/RConn1
  220_kV_Kondelwald;_220kV_Wengerohr_CN_66764943_220000_CN_152107815_220000/RConn2 -- T_152107815_220000;110000_Otterbach/LConn2 -- _CN_152107815_220000_CN_152022992_220000/RConn2
  220_kV_Kondelwald;_220kV_Wengerohr_CN_66764943_220000_CN_152107815_220000/RConn3 -- T_152107815_220000;110000_Otterbach/LConn3 -- _CN_152107815_220000_CN_152022992_220000/RConn3
  220_kV_Kondelwald;_220kV_Wengerohr_CN_66764943_220000_CN_151967290_220000/RConn1 -- T_151967290_380000;220000;110000_Station_Niederstedem/RConn1 -- _CN_89176939_220000_CN_151967290_220000/LConn1 -- L_151967290/LConn1
  220_kV_Kondelwald;_220kV_Wengerohr_CN_66764943_220000_CN_151967290_220000/RConn2 -- T_151967290_380000;220000;110000_Station_Niederstedem/RConn2 -- _CN_89176939_220000_CN_151967290_220000/LConn2 -- L_151967290/LConn2
  220_kV_Kondelwald;_220kV_Wengerohr_CN_66764943_220000_CN_151967290_220000/RConn3 -- T_151967290_380000;220000;110000_Station_Niederstedem/RConn3 -- _CN_89176939_220000_CN_151967290_220000/LConn3 -- L_151967290/LConn3
  220_kV_Kondelwald;_220kV_Wengerohr_CN_66764943_220000_CN_395847307_220000/RConn1 -- T_395847307_380000;220000;110000_Station_Weißenthurm/RConn1 -- 220_kV_Berggeist_West;_Nette_Ost_CN_42423415_220000_CN_395847307_220000/LConn1 -- _CN_154869247_220000_CN_395847307_220000/LConn1 -- L_395847307/LConn1
  220_kV_Kondelwald;_220kV_Wengerohr_CN_66764943_220000_CN_395847307_220000/RConn2 -- T_395847307_380000;220000;110000_Station_Weißenthurm/RConn2 -- 220_kV_Berggeist_West;_Nette_Ost_CN_42423415_220000_CN_395847307_220000/LConn2 -- _CN_154869247_220000_CN_395847307_220000/LConn2 -- L_395847307/LConn2
  220_kV_Kondelwald;_220kV_Wengerohr_CN_66764943_220000_CN_395847307_220000/RConn3 -- T_395847307_380000;220000;110000_Station_Weißenthurm/RConn3 -- 220_kV_Berggeist_West;_Nette_Ost_CN_42423415_220000_CN_395847307_220000/LConn3 -- _CN_154869247_220000_CN_395847307_220000/LConn3 -- L_395847307/LConn3
  _CN_24268944_380000_CN_26593929_380000/LConn1 -- T_24268944_380000;110000_Station_Verlautenheide/LConn1 -- _CN_24268944_380000_CN11346170/LConn1 -- _CN_24268944_380000_CN_25426571_380000/LConn1
  _CN_24268944_380000_CN_26593929_380000/LConn2 -- T_24268944_380000;110000_Station_Verlautenheide/LConn2 -- _CN_24268944_380000_CN11346170/LConn2 -- _CN_24268944_380000_CN_25426571_380000/LConn2
  _CN_24268944_380000_CN_26593929_380000/LConn3 -- T_24268944_380000;110000_Station_Verlautenheide/LConn3 -- _CN_24268944_380000_CN11346170/LConn3 -- _CN_24268944_380000_CN_25426571_380000/LConn3
  _CN_24268944_380000_CN_26593929_380000/RConn1 -- T_26593929_380000;110000_Station_Oberzier/LConn1 -- _CN_25992879_380000_CN_26593929_380000/LConn1 -- 380_kV_Oberzier_Süd;_Selfkant_weiss_CN_26927264_380000_CN_26593929_380000/LConn1 -- 380_kV_Sechtem_Nord|Süd;_Walberberg_West_CN_22766160_380000_CN_26593929_380000/LConn1 -- _CN_26593935_380000_CN_26593929_380000/LConn1 -- _CN_151967290_380000_CN_26593929_380000/LConn1
  _CN_24268944_380000_CN_26593929_380000/RConn2 -- T_26593929_380000;110000_Station_Oberzier/LConn2 -- _CN_25992879_380000_CN_26593929_380000/LConn2 -- 380_kV_Oberzier_Süd;_Selfkant_weiss_CN_26927264_380000_CN_26593929_380000/LConn2 -- 380_kV_Sechtem_Nord|Süd;_Walberberg_West_CN_22766160_380000_CN_26593929_380000/LConn2 -- _CN_26593935_380000_CN_26593929_380000/LConn2 -- _CN_151967290_380000_CN_26593929_380000/LConn2
  _CN_24268944_380000_CN_26593929_380000/RConn3 -- T_26593929_380000;110000_Station_Oberzier/LConn3 -- _CN_25992879_380000_CN_26593929_380000/LConn3 -- 380_kV_Oberzier_Süd;_Selfkant_weiss_CN_26927264_380000_CN_26593929_380000/LConn3 -- 380_kV_Sechtem_Nord|Süd;_Walberberg_West_CN_22766160_380000_CN_26593929_380000/LConn3 -- _CN_26593935_380000_CN_26593929_380000/LConn3 -- _CN_151967290_380000_CN_26593929_380000/LConn3
  G_11346170_RWE_Kraftwerk_Weisweiler/RConn1 -- _CN_24268944_380000_CN11346170/RConn1
  G_11346170_RWE_Kraftwerk_Weisweiler/RConn2 -- _CN_24268944_380000_CN11346170/RConn2
  G_11346170_RWE_Kraftwerk_Weisweiler/RConn3 -- _CN_24268944_380000_CN11346170/RConn3
  T_25426571_380000;110000_Umspannwerk_Weisweiler/LConn1 -- _CN_24268944_380000_CN_25426571_380000/RConn1
  T_25426571_380000;110000_Umspannwerk_Weisweiler/LConn2 -- _CN_24268944_380000_CN_25426571_380000/RConn2
  T_25426571_380000;110000_Umspannwerk_Weisweiler/LConn3 -- _CN_24268944_380000_CN_25426571_380000/RConn3
  _CN_89215122_220000_CN_82310607_220000/LConn1 -- T_89215122_220000;110000_Station_Saarwellingen/LConn1 -- _CN_89215122_220000_CN_54359256_220000/RConn1 -- _CN_89215122_220000_CN_145680894_220000/RConn1
  _CN_89215122_220000_CN_82310607_220000/LConn2 -- T_89215122_220000;110000_Station_Saarwellingen/LConn2 -- _CN_89215122_220000_CN_54359256_220000/RConn2 -- _CN_89215122_220000_CN_145680894_220000/RConn2
  _CN_89215122_220000_CN_82310607_220000/LConn3 -- T_89215122_220000;110000_Station_Saarwellingen/LConn3 -- _CN_89215122_220000_CN_54359256_220000/RConn3 -- _CN_89215122_220000_CN_145680894_220000/RConn3
  _CN_89215122_220000_CN_82310607_220000/RConn1 -- T_82310607_220000_Dieffeln/LConn1 -- _CN_90109302_220000_CN_82310607_220000/LConn1 -- _CN_82310607_220000_CN_90109304_220000/LConn1
  _CN_89215122_220000_CN_82310607_220000/RConn2 -- T_82310607_220000_Dieffeln/LConn2 -- _CN_90109302_220000_CN_82310607_220000/LConn2 -- _CN_82310607_220000_CN_90109304_220000/LConn2
  _CN_89215122_220000_CN_82310607_220000/RConn3 -- T_82310607_220000_Dieffeln/LConn3 -- _CN_90109302_220000_CN_82310607_220000/LConn3 -- _CN_82310607_220000_CN_90109304_220000/LConn3
  3105_CN_24502420_380000_CN275650140/RConn1 -- G_275650140_Kernkraftwerk_Brokdorf/RConn1 -- 202_UW_HH_Nord_UW_Itzehoe_West_CN_60032354_220000_CN275650140/LConn1
  3105_CN_24502420_380000_CN275650140/RConn2 -- G_275650140_Kernkraftwerk_Brokdorf/RConn2 -- 202_UW_HH_Nord_UW_Itzehoe_West_CN_60032354_220000_CN275650140/LConn2
  3105_CN_24502420_380000_CN275650140/RConn3 -- G_275650140_Kernkraftwerk_Brokdorf/RConn3 -- 202_UW_HH_Nord_UW_Itzehoe_West_CN_60032354_220000_CN275650140/LConn3
  T_31927411_380000;110000_Alfstedt/LConn1 -- _CN_24502420_380000_CN_31927411_380000/RConn1
  T_31927411_380000;110000_Alfstedt/LConn2 -- _CN_24502420_380000_CN_31927411_380000/RConn2
  T_31927411_380000;110000_Alfstedt/LConn3 -- _CN_24502420_380000_CN_31927411_380000/RConn3
  F_CN_24502420_380000_CN_11285720_380000/RConn1 -- T_11285720_380000;110000_Umspannwerk_Hamburg_Süd/LConn1 -- D_CN_23583867_380000_CN_11285720_380000/RConn1 -- _CN_11285720_380000_CN101400025/LConn1
  F_CN_24502420_380000_CN_11285720_380000/RConn2 -- T_11285720_380000;110000_Umspannwerk_Hamburg_Süd/LConn2 -- D_CN_23583867_380000_CN_11285720_380000/RConn2 -- _CN_11285720_380000_CN101400025/LConn2
  F_CN_24502420_380000_CN_11285720_380000/RConn3 -- T_11285720_380000;110000_Umspannwerk_Hamburg_Süd/LConn3 -- D_CN_23583867_380000_CN_11285720_380000/RConn3 -- _CN_11285720_380000_CN101400025/LConn3
  380_kV_Leichlingen_West_CN_33816726_380000_CN_22761839_380000/LConn1 -- T_33816726_380000;110000_Station_Halfeshof/LConn1 -- 380_kV_Leichlingen_West_CN_33816726_380000_CN_152403632_380000/LConn1 -- 380_kV_Leichlingen_West_CN_33816726_380000_CN_92165128_380000/LConn1
  380_kV_Leichlingen_West_CN_33816726_380000_CN_22761839_380000/LConn2 -- T_33816726_380000;110000_Station_Halfeshof/LConn2 -- 380_kV_Leichlingen_West_CN_33816726_380000_CN_152403632_380000/LConn2 -- 380_kV_Leichlingen_West_CN_33816726_380000_CN_92165128_380000/LConn2
  380_kV_Leichlingen_West_CN_33816726_380000_CN_22761839_380000/LConn3 -- T_33816726_380000;110000_Station_Halfeshof/LConn3 -- 380_kV_Leichlingen_West_CN_33816726_380000_CN_152403632_380000/LConn3 -- 380_kV_Leichlingen_West_CN_33816726_380000_CN_92165128_380000/LConn3
  380_kV_Leichlingen_West_CN_33816726_380000_CN_22761839_380000/RConn1 -- T_22761839_380000;220000;110000_Station_Opladen/LConn1 -- 380_kV_Neurath_2b;_Oerkhaus_Ost_CN_22761839_380000_CN_49577448_380000/LConn1 -- 380_kV_Neurath_2b;_Oerkhaus_Ost_CN_22761839_380000_CN_106096507_380000/LConn1 -- 380_kV_Neurath_2b;_Oerkhaus_Ost_CN_22761839_380000_CN_113546939_380000/RConn1 -- 380_kV_Opladen_Nord|Süd_CN_22761839_380000_CN_24839976_380000/LConn1
  380_kV_Leichlingen_West_CN_33816726_380000_CN_22761839_380000/RConn2 -- T_22761839_380000;220000;110000_Station_Opladen/LConn2 -- 380_kV_Neurath_2b;_Oerkhaus_Ost_CN_22761839_380000_CN_49577448_380000/LConn2 -- 380_kV_Neurath_2b;_Oerkhaus_Ost_CN_22761839_380000_CN_106096507_380000/LConn2 -- 380_kV_Neurath_2b;_Oerkhaus_Ost_CN_22761839_380000_CN_113546939_380000/RConn2 -- 380_kV_Opladen_Nord|Süd_CN_22761839_380000_CN_24839976_380000/LConn2
  380_kV_Leichlingen_West_CN_33816726_380000_CN_22761839_380000/RConn3 -- T_22761839_380000;220000;110000_Station_Opladen/LConn3 -- 380_kV_Neurath_2b;_Oerkhaus_Ost_CN_22761839_380000_CN_49577448_380000/LConn3 -- 380_kV_Neurath_2b;_Oerkhaus_Ost_CN_22761839_380000_CN_106096507_380000/LConn3 -- 380_kV_Neurath_2b;_Oerkhaus_Ost_CN_22761839_380000_CN_113546939_380000/RConn3 -- 380_kV_Opladen_Nord|Süd_CN_22761839_380000_CN_24839976_380000/LConn3
  380_kV_Leichlingen_West_CN_33816726_380000_CN_152403632_380000/RConn1 -- T_152403632_380000;220000;110000_Station_Dauersberg/LConn1 -- _CN_24536211_380000_CN_152403632_380000/LConn1 -- 380kV_Limburg_West_CN_50898216_380000_CN_152403632_380000/LConn1 -- 380_kV_Siegtal_Nord|Süd_CN_22766160_380000_CN_152403632_380000/LConn1
  380_kV_Leichlingen_West_CN_33816726_380000_CN_152403632_380000/RConn2 -- T_152403632_380000;220000;110000_Station_Dauersberg/LConn2 -- _CN_24536211_380000_CN_152403632_380000/LConn2 -- 380kV_Limburg_West_CN_50898216_380000_CN_152403632_380000/LConn2 -- 380_kV_Siegtal_Nord|Süd_CN_22766160_380000_CN_152403632_380000/LConn2
  380_kV_Leichlingen_West_CN_33816726_380000_CN_152403632_380000/RConn3 -- T_152403632_380000;220000;110000_Station_Dauersberg/LConn3 -- _CN_24536211_380000_CN_152403632_380000/LConn3 -- 380kV_Limburg_West_CN_50898216_380000_CN_152403632_380000/LConn3 -- 380_kV_Siegtal_Nord|Süd_CN_22766160_380000_CN_152403632_380000/LConn3
  T_92165128_380000;110000_Station_Linde/LConn1 -- 380_kV_Leichlingen_West_CN_33816726_380000_CN_92165128_380000/RConn1
  T_92165128_380000;110000_Station_Linde/LConn2 -- 380_kV_Leichlingen_West_CN_33816726_380000_CN_92165128_380000/RConn2
  T_92165128_380000;110000_Station_Linde/LConn3 -- 380_kV_Leichlingen_West_CN_33816726_380000_CN_92165128_380000/RConn3
  T_32731290_220000;110000_Karlsruhe_West/LConn1 -- Daxlanden___Mühlburg_CN_32731290_220000_CN_152261133_220000/RConn1
  T_32731290_220000;110000_Karlsruhe_West/LConn2 -- Daxlanden___Mühlburg_CN_32731290_220000_CN_152261133_220000/RConn2
  T_32731290_220000;110000_Karlsruhe_West/LConn3 -- Daxlanden___Mühlburg_CN_32731290_220000_CN_152261133_220000/RConn3
  380_kV_Paffendorf_Süd;_Selfkant_weiß_CN_26927264_380000_CN_24839976_380000/LConn1 -- T_26927264_380000;110000_Station_Paffendorf/LConn1 -- 380_kV_Oberzier_Süd;_Selfkant_weiss_CN_26927264_380000_CN_26593929_380000/RConn1
  380_kV_Paffendorf_Süd;_Selfkant_weiß_CN_26927264_380000_CN_24839976_380000/LConn2 -- T_26927264_380000;110000_Station_Paffendorf/LConn2 -- 380_kV_Oberzier_Süd;_Selfkant_weiss_CN_26927264_380000_CN_26593929_380000/RConn2
  380_kV_Paffendorf_Süd;_Selfkant_weiß_CN_26927264_380000_CN_24839976_380000/LConn3 -- T_26927264_380000;110000_Station_Paffendorf/LConn3 -- 380_kV_Oberzier_Süd;_Selfkant_weiss_CN_26927264_380000_CN_26593929_380000/RConn3
  380_kV_Paffendorf_Süd;_Selfkant_weiß_CN_26927264_380000_CN_24839976_380000/RConn1 -- T_24839976_380000;220000_Umspannwerk_Rommerskirchen/LConn1 -- _CN_24839976_380000_CN24840439/LConn1 -- 380_kV_Opladen_Nord|Süd_CN_22761839_380000_CN_24839976_380000/RConn1 -- 380kV_Knechtsteden_West_CN_77179271_380000_CN_24839976_380000/LConn1 -- 380_kV_Ville_Ost_CN_22766160_380000_CN_24839976_380000/LConn1
  380_kV_Paffendorf_Süd;_Selfkant_weiß_CN_26927264_380000_CN_24839976_380000/RConn2 -- T_24839976_380000;220000_Umspannwerk_Rommerskirchen/LConn2 -- _CN_24839976_380000_CN24840439/LConn2 -- 380_kV_Opladen_Nord|Süd_CN_22761839_380000_CN_24839976_380000/RConn2 -- 380kV_Knechtsteden_West_CN_77179271_380000_CN_24839976_380000/LConn2 -- 380_kV_Ville_Ost_CN_22766160_380000_CN_24839976_380000/LConn2
  380_kV_Paffendorf_Süd;_Selfkant_weiß_CN_26927264_380000_CN_24839976_380000/RConn3 -- T_24839976_380000;220000_Umspannwerk_Rommerskirchen/LConn3 -- _CN_24839976_380000_CN24840439/LConn3 -- 380_kV_Opladen_Nord|Süd_CN_22761839_380000_CN_24839976_380000/RConn3 -- 380kV_Knechtsteden_West_CN_77179271_380000_CN_24839976_380000/LConn3 -- 380_kV_Ville_Ost_CN_22766160_380000_CN_24839976_380000/LConn3
  _CN_23406775_380000_CN401876926/LConn1 -- T_23406775_380000;110000_Pulgar/LConn1 -- _CN_23406775_380000_CN_32843531_380000/LConn1 -- _CN_23406775_380000_CN_143882655_380000/LConn1
  _CN_23406775_380000_CN401876926/LConn2 -- T_23406775_380000;110000_Pulgar/LConn2 -- _CN_23406775_380000_CN_32843531_380000/LConn2 -- _CN_23406775_380000_CN_143882655_380000/LConn2
  _CN_23406775_380000_CN401876926/LConn3 -- T_23406775_380000;110000_Pulgar/LConn3 -- _CN_23406775_380000_CN_32843531_380000/LConn3 -- _CN_23406775_380000_CN_143882655_380000/LConn3
  G_401876926_Kraftwerk_Lippendorf/RConn1 -- _CN_23406775_380000_CN401876926/RConn1
  G_401876926_Kraftwerk_Lippendorf/RConn2 -- _CN_23406775_380000_CN401876926/RConn2
  G_401876926_Kraftwerk_Lippendorf/RConn3 -- _CN_23406775_380000_CN401876926/RConn3
  _CN_23406775_380000_CN_143882655_380000/RConn1 -- T_143882655_380000;220000;110000_Umspannwerk_Vieselbach/LConn1 -- _CN_143882655_380000_CN_148211527_380000/LConn1 -- _CN_143882655_380000_CN_128277645_380000/LConn1 -- _CN_143882655_380000_CN_29713902_380000/LConn1 -- _CN_143882655_380000_CN_29309786_380000/LConn1 -- _CN_143882655_380000_CN_154418450_380000/LConn1 -- 467_CN_149256409_380000_CN_143882655_380000/LConn1
  _CN_23406775_380000_CN_143882655_380000/RConn2 -- T_143882655_380000;220000;110000_Umspannwerk_Vieselbach/LConn2 -- _CN_143882655_380000_CN_148211527_380000/LConn2 -- _CN_143882655_380000_CN_128277645_380000/LConn2 -- _CN_143882655_380000_CN_29713902_380000/LConn2 -- _CN_143882655_380000_CN_29309786_380000/LConn2 -- _CN_143882655_380000_CN_154418450_380000/LConn2 -- 467_CN_149256409_380000_CN_143882655_380000/LConn2
  _CN_23406775_380000_CN_143882655_380000/RConn3 -- T_143882655_380000;220000;110000_Umspannwerk_Vieselbach/LConn3 -- _CN_143882655_380000_CN_148211527_380000/LConn3 -- _CN_143882655_380000_CN_128277645_380000/LConn3 -- _CN_143882655_380000_CN_29713902_380000/LConn3 -- _CN_143882655_380000_CN_29309786_380000/LConn3 -- _CN_143882655_380000_CN_154418450_380000/LConn3 -- 467_CN_149256409_380000_CN_143882655_380000/LConn3
  _CN_23406775_380000_CN_32843531_380000/RConn1 -- T_32843531_380000;220000;110000_Eula/LConn1 -- 585_CN_157328339_380000_CN_32843531_380000/LConn1
  _CN_23406775_380000_CN_32843531_380000/RConn2 -- T_32843531_380000;220000;110000_Eula/LConn2 -- 585_CN_157328339_380000_CN_32843531_380000/LConn2
  _CN_23406775_380000_CN_32843531_380000/RConn3 -- T_32843531_380000;220000;110000_Eula/LConn3 -- 585_CN_157328339_380000_CN_32843531_380000/LConn3
  Oberbachern___Neufinsing_CN_24158385_220000_CN_18629425_220000/RConn1 -- T_18629425_380000;220000;110000_Umspannwerk_Oberbachern/RConn1 -- Oberbrunn___Oberbachern_CN_18629425_220000_CN_24237879_220000/LConn1 -- L_18629425/LConn1
  Oberbachern___Neufinsing_CN_24158385_220000_CN_18629425_220000/RConn2 -- T_18629425_380000;220000;110000_Umspannwerk_Oberbachern/RConn2 -- Oberbrunn___Oberbachern_CN_18629425_220000_CN_24237879_220000/LConn2 -- L_18629425/LConn2
  Oberbachern___Neufinsing_CN_24158385_220000_CN_18629425_220000/RConn3 -- T_18629425_380000;220000;110000_Umspannwerk_Oberbachern/RConn3 -- Oberbrunn___Oberbachern_CN_18629425_220000_CN_24237879_220000/LConn3 -- L_18629425/LConn3
  Neufinsing___Zolling_CN_24158385_220000_CN_133342285_220000/RConn1 -- T_133342285_220000;110000_Zolling___Irsching/LConn1 -- _CN_232833796_220000_CN_133342285_220000/LConn1
  Neufinsing___Zolling_CN_24158385_220000_CN_133342285_220000/RConn2 -- T_133342285_220000;110000_Zolling___Irsching/LConn2 -- _CN_232833796_220000_CN_133342285_220000/LConn2
  Neufinsing___Zolling_CN_24158385_220000_CN_133342285_220000/RConn3 -- T_133342285_220000;110000_Zolling___Irsching/LConn3 -- _CN_232833796_220000_CN_133342285_220000/LConn3
  T_75865676_220000_Umspannwerk_Marienberg/LConn1 -- _CN_24158385_220000_CN_75865676_220000/RConn1
  T_75865676_220000_Umspannwerk_Marienberg/LConn2 -- _CN_24158385_220000_CN_75865676_220000/RConn2
  T_75865676_220000_Umspannwerk_Marienberg/LConn3 -- _CN_24158385_220000_CN_75865676_220000/RConn3
  T_154110133_380000_/LConn1 -- _CN_154110133_380000_CN161909939/LConn1
  T_154110133_380000_/LConn2 -- _CN_154110133_380000_CN161909939/LConn2
  T_154110133_380000_/LConn3 -- _CN_154110133_380000_CN161909939/LConn3
  _CN_154110133_380000_CN161909939/RConn1 -- G_161909939_Kernkraftwerk_Philippsburg/RConn1 -- Elsenz_CN_143903369_380000_CN161909939/LConn1 -- Philippsburg___Pulverdingen_CN_43688805_380000_CN161909939/LConn1 -- Daxlanden___Philippsburg_CN_154110135_380000_CN161909939/LConn1 -- _CN_152261133_380000_CN161909939/RConn1
  _CN_154110133_380000_CN161909939/RConn2 -- G_161909939_Kernkraftwerk_Philippsburg/RConn2 -- Elsenz_CN_143903369_380000_CN161909939/LConn2 -- Philippsburg___Pulverdingen_CN_43688805_380000_CN161909939/LConn2 -- Daxlanden___Philippsburg_CN_154110135_380000_CN161909939/LConn2 -- _CN_152261133_380000_CN161909939/RConn2
  _CN_154110133_380000_CN161909939/RConn3 -- G_161909939_Kernkraftwerk_Philippsburg/RConn3 -- Elsenz_CN_143903369_380000_CN161909939/LConn3 -- Philippsburg___Pulverdingen_CN_43688805_380000_CN161909939/LConn3 -- Daxlanden___Philippsburg_CN_154110135_380000_CN161909939/LConn3 -- _CN_152261133_380000_CN161909939/RConn3
  T_90109302_220000_UA_Obergraben/LConn1 -- _CN_90109302_220000_CN_82310607_220000/RConn1
  T_90109302_220000_UA_Obergraben/LConn2 -- _CN_90109302_220000_CN_82310607_220000/RConn2
  T_90109302_220000_UA_Obergraben/LConn3 -- _CN_90109302_220000_CN_82310607_220000/RConn3
  A08___A09_CN_28397771_220000_CN_23135618_220000/LConn1 -- T_28397771_220000;110000_UW_Veltheim/LConn1 -- _CN_28397771_220000_CN149331961/LConn1 -- _CN_28397771_220000_CN_26611458_220000/LConn1 -- _CN_28397771_220000_CN_24264701_220000/LConn1 -- _CN_28397771_220000_CN_288305056_220000/LConn1
  A08___A09_CN_28397771_220000_CN_23135618_220000/LConn2 -- T_28397771_220000;110000_UW_Veltheim/LConn2 -- _CN_28397771_220000_CN149331961/LConn2 -- _CN_28397771_220000_CN_26611458_220000/LConn2 -- _CN_28397771_220000_CN_24264701_220000/LConn2 -- _CN_28397771_220000_CN_288305056_220000/LConn2
  A08___A09_CN_28397771_220000_CN_23135618_220000/LConn3 -- T_28397771_220000;110000_UW_Veltheim/LConn3 -- _CN_28397771_220000_CN149331961/LConn3 -- _CN_28397771_220000_CN_26611458_220000/LConn3 -- _CN_28397771_220000_CN_24264701_220000/LConn3 -- _CN_28397771_220000_CN_288305056_220000/LConn3
  T_23135618_220000;110000_Umspannwerk_Meißen/LConn1 -- A08___A09_CN_28397771_220000_CN_23135618_220000/RConn1
  T_23135618_220000;110000_Umspannwerk_Meißen/LConn2 -- A08___A09_CN_28397771_220000_CN_23135618_220000/RConn2
  T_23135618_220000;110000_Umspannwerk_Meißen/LConn3 -- A08___A09_CN_28397771_220000_CN_23135618_220000/RConn3
  G_149331961_Gemeinschaftskraftwerk_Veltheim/RConn1 -- _CN_28397771_220000_CN149331961/RConn1
  G_149331961_Gemeinschaftskraftwerk_Veltheim/RConn2 -- _CN_28397771_220000_CN149331961/RConn2
  G_149331961_Gemeinschaftskraftwerk_Veltheim/RConn3 -- _CN_28397771_220000_CN149331961/RConn3
  _CN_28397771_220000_CN_26611458_220000/RConn1 -- T_26611458_220000;110000_Umspannwerk_Bielefeld_Ost/LConn1 -- _CN_26383042_220000_CN_26611458_220000/LConn1
  _CN_28397771_220000_CN_26611458_220000/RConn2 -- T_26611458_220000;110000_Umspannwerk_Bielefeld_Ost/LConn2 -- _CN_26383042_220000_CN_26611458_220000/LConn2
  _CN_28397771_220000_CN_26611458_220000/RConn3 -- T_26611458_220000;110000_Umspannwerk_Bielefeld_Ost/LConn3 -- _CN_26383042_220000_CN_26611458_220000/LConn3
  _CN_28397771_220000_CN_24264701_220000/RConn1 -- T_24264701_380000;220000;110000_Umspannwerk_Bechterdissen/RConn1 -- _CN_158253525_220000_CN_24264701_220000/LConn1 -- L_24264701/LConn1
  _CN_28397771_220000_CN_24264701_220000/RConn2 -- T_24264701_380000;220000;110000_Umspannwerk_Bechterdissen/RConn2 -- _CN_158253525_220000_CN_24264701_220000/LConn2 -- L_24264701/LConn2
  _CN_28397771_220000_CN_24264701_220000/RConn3 -- T_24264701_380000;220000;110000_Umspannwerk_Bechterdissen/RConn3 -- _CN_158253525_220000_CN_24264701_220000/LConn3 -- L_24264701/LConn3
  T_288305056_220000;110000_Umspannwerk_Lage/LConn1 -- _CN_28397771_220000_CN_288305056_220000/RConn1
  T_288305056_220000;110000_Umspannwerk_Lage/LConn2 -- _CN_28397771_220000_CN_288305056_220000/RConn2
  T_288305056_220000;110000_Umspannwerk_Lage/LConn3 -- _CN_28397771_220000_CN_288305056_220000/RConn3
  Altenfeld___Redwitz_CN_149256409_380000_CN_24757392_380000/RConn1 -- T_149256409_380000;110000_Umspannwerk_Altenfeld/LConn1 -- _CN_149256409_380000_CN_128277645_380000/LConn1 -- 467_CN_149256409_380000_CN_143882655_380000/RConn1 -- Altenfeld___Redwitz_CN_149256409_380000_CN_25746125_380000/LConn1
  Altenfeld___Redwitz_CN_149256409_380000_CN_24757392_380000/RConn2 -- T_149256409_380000;110000_Umspannwerk_Altenfeld/LConn2 -- _CN_149256409_380000_CN_128277645_380000/LConn2 -- 467_CN_149256409_380000_CN_143882655_380000/RConn2 -- Altenfeld___Redwitz_CN_149256409_380000_CN_25746125_380000/LConn2
  Altenfeld___Redwitz_CN_149256409_380000_CN_24757392_380000/RConn3 -- T_149256409_380000;110000_Umspannwerk_Altenfeld/LConn3 -- _CN_149256409_380000_CN_128277645_380000/LConn3 -- 467_CN_149256409_380000_CN_143882655_380000/RConn3 -- Altenfeld___Redwitz_CN_149256409_380000_CN_25746125_380000/LConn3
  T_25746125_380000_Pumpspeicherwerk_Goldisthal/LConn1 -- Altenfeld___Redwitz_CN_149256409_380000_CN_25746125_380000/RConn1
  T_25746125_380000_Pumpspeicherwerk_Goldisthal/LConn2 -- Altenfeld___Redwitz_CN_149256409_380000_CN_25746125_380000/RConn2
  T_25746125_380000_Pumpspeicherwerk_Goldisthal/LConn3 -- Altenfeld___Redwitz_CN_149256409_380000_CN_25746125_380000/RConn3
  _CN_149256409_380000_CN_128277645_380000/RConn1 -- T_128277645_380000;220000;110000_Umspannwerk_Remptendorf/LConn1 -- 574_Remptendorf___Röhrsdorf;_573_Remptendorf___Weida_CN_128277645_380000_CN_156673637_380000/LConn1 -- 574_Remptendorf___Röhrsdorf;_573_Remptendorf___Weida_CN_128277645_380000_CN_23117075_380000/RConn1 -- _CN_143882655_380000_CN_128277645_380000/RConn1 -- _CN_128277645_380000_CN_24757392_380000/RConn1
  _CN_149256409_380000_CN_128277645_380000/RConn2 -- T_128277645_380000;220000;110000_Umspannwerk_Remptendorf/LConn2 -- 574_Remptendorf___Röhrsdorf;_573_Remptendorf___Weida_CN_128277645_380000_CN_156673637_380000/LConn2 -- 574_Remptendorf___Röhrsdorf;_573_Remptendorf___Weida_CN_128277645_380000_CN_23117075_380000/RConn2 -- _CN_143882655_380000_CN_128277645_380000/RConn2 -- _CN_128277645_380000_CN_24757392_380000/RConn2
  _CN_149256409_380000_CN_128277645_380000/RConn3 -- T_128277645_380000;220000;110000_Umspannwerk_Remptendorf/LConn3 -- 574_Remptendorf___Röhrsdorf;_573_Remptendorf___Weida_CN_128277645_380000_CN_156673637_380000/LConn3 -- 574_Remptendorf___Röhrsdorf;_573_Remptendorf___Weida_CN_128277645_380000_CN_23117075_380000/RConn3 -- _CN_143882655_380000_CN_128277645_380000/RConn3 -- _CN_128277645_380000_CN_24757392_380000/RConn3
  T_150200540_220000_Kraftwerkschaltanlage_Ibbenbüren/LConn1 -- _CN_150200540_220000_CN196878039/LConn1
  T_150200540_220000_Kraftwerkschaltanlage_Ibbenbüren/LConn2 -- _CN_150200540_220000_CN196878039/LConn2
  T_150200540_220000_Kraftwerkschaltanlage_Ibbenbüren/LConn3 -- _CN_150200540_220000_CN196878039/LConn3
  _CN_150200540_220000_CN196878039/RConn1 -- G_196878039_RWE_Power_AG_Kraftwerk_Ibbenbüren/RConn1 -- 220kV_Ibbenbüren_B_CN_114319248_220000_CN196878039/RConn1
  _CN_150200540_220000_CN196878039/RConn2 -- G_196878039_RWE_Power_AG_Kraftwerk_Ibbenbüren/RConn2 -- 220kV_Ibbenbüren_B_CN_114319248_220000_CN196878039/RConn2
  _CN_150200540_220000_CN196878039/RConn3 -- G_196878039_RWE_Power_AG_Kraftwerk_Ibbenbüren/RConn3 -- 220kV_Ibbenbüren_B_CN_114319248_220000_CN196878039/RConn3
  220kV_Walsum_Süd_CN_37554416_220000_CN_35833592_220000/LConn1 -- T_37554416_220000;110000_Station_Hamborn/LConn1 -- 220kV_Dinslaken_West_CN_37554416_220000_CN_24921206_220000/LConn1 -- 220kV_Dinslaken_West_CN_37554416_220000_CN_25032036_220000/LConn1 -- 220kV_Walsum_Süd_CN_37554416_220000_CN_35818137_220000/LConn1 -- 220kV_Walsum_Süd_CN_37554416_220000_CN26623135/LConn1 -- 220kV_Dinslaken_West_CN_37554416_220000_CN_24462426_220000/LConn1 -- 220kV_Dinslaken_West_CN_37554416_220000_CN_46852069_220000/LConn1
  220kV_Walsum_Süd_CN_37554416_220000_CN_35833592_220000/LConn2 -- T_37554416_220000;110000_Station_Hamborn/LConn2 -- 220kV_Dinslaken_West_CN_37554416_220000_CN_24921206_220000/LConn2 -- 220kV_Dinslaken_West_CN_37554416_220000_CN_25032036_220000/LConn2 -- 220kV_Walsum_Süd_CN_37554416_220000_CN_35818137_220000/LConn2 -- 220kV_Walsum_Süd_CN_37554416_220000_CN26623135/LConn2 -- 220kV_Dinslaken_West_CN_37554416_220000_CN_24462426_220000/LConn2 -- 220kV_Dinslaken_West_CN_37554416_220000_CN_46852069_220000/LConn2
  220kV_Walsum_Süd_CN_37554416_220000_CN_35833592_220000/LConn3 -- T_37554416_220000;110000_Station_Hamborn/LConn3 -- 220kV_Dinslaken_West_CN_37554416_220000_CN_24921206_220000/LConn3 -- 220kV_Dinslaken_West_CN_37554416_220000_CN_25032036_220000/LConn3 -- 220kV_Walsum_Süd_CN_37554416_220000_CN_35818137_220000/LConn3 -- 220kV_Walsum_Süd_CN_37554416_220000_CN26623135/LConn3 -- 220kV_Dinslaken_West_CN_37554416_220000_CN_24462426_220000/LConn3 -- 220kV_Dinslaken_West_CN_37554416_220000_CN_46852069_220000/LConn3
  220kV_Walsum_Süd_CN_37554416_220000_CN_35833592_220000/RConn1 -- T_35833592_220000_/LConn1 -- _CN_35833592_220000_CN_35833442_220000/LConn1
  220kV_Walsum_Süd_CN_37554416_220000_CN_35833592_220000/RConn2 -- T_35833592_220000_/LConn2 -- _CN_35833592_220000_CN_35833442_220000/LConn2
  220kV_Walsum_Süd_CN_37554416_220000_CN_35833592_220000/RConn3 -- T_35833592_220000_/LConn3 -- _CN_35833592_220000_CN_35833442_220000/LConn3
  220kV_Walsum_Süd_CN_37554416_220000_CN_35818137_220000/RConn1 -- T_35818137_380000;220000;110000_Station_Beeck/RConn1 -- Stockum_Ost+West_CN_35818134_220000_CN_35818137_220000/LConn1 -- _CN_35818137_220000_CN_35818522_220000/LConn1 -- L_35818137/LConn1
  220kV_Walsum_Süd_CN_37554416_220000_CN_35818137_220000/RConn2 -- T_35818137_380000;220000;110000_Station_Beeck/RConn2 -- Stockum_Ost+West_CN_35818134_220000_CN_35818137_220000/LConn2 -- _CN_35818137_220000_CN_35818522_220000/LConn2 -- L_35818137/LConn2
  220kV_Walsum_Süd_CN_37554416_220000_CN_35818137_220000/RConn3 -- T_35818137_380000;220000;110000_Station_Beeck/RConn3 -- Stockum_Ost+West_CN_35818134_220000_CN_35818137_220000/LConn3 -- _CN_35818137_220000_CN_35818522_220000/LConn3 -- L_35818137/LConn3
  220kV_Walsum_Süd_CN_37554416_220000_CN26623135/RConn1 -- G_26623135_Kraftwerk_Duisburg_Walsum/RConn1 -- 380kV_Lohheide_West_CN_23380800_380000_CN26623135/LConn1 -- 220kV_Beeck_Tr211+212_CN_24478889_220000_CN26623135/LConn1 -- _CN_76185022_380000_CN26623135/LConn1
  220kV_Walsum_Süd_CN_37554416_220000_CN26623135/RConn2 -- G_26623135_Kraftwerk_Duisburg_Walsum/RConn2 -- 380kV_Lohheide_West_CN_23380800_380000_CN26623135/LConn2 -- 220kV_Beeck_Tr211+212_CN_24478889_220000_CN26623135/LConn2 -- _CN_76185022_380000_CN26623135/LConn2
  220kV_Walsum_Süd_CN_37554416_220000_CN26623135/RConn3 -- G_26623135_Kraftwerk_Duisburg_Walsum/RConn3 -- 380kV_Lohheide_West_CN_23380800_380000_CN26623135/LConn3 -- 220kV_Beeck_Tr211+212_CN_24478889_220000_CN26623135/LConn3 -- _CN_76185022_380000_CN26623135/LConn3
  220kV_Dinslaken_West_CN_37554416_220000_CN_24462426_220000/RConn1 -- T_24462426_380000;220000;110000_Station_Niederrhein/RConn1 -- _CN_24462426_220000_CN_23084417_220000/LConn1 -- L_24462426/LConn1 -- 220kV_Scholven_E_CN_23022100_220000_CN_24462426_220000/RConn1 -- 220kV_Wesel_Ost_CN_24462426_220000_CN_23380800_220000/LConn1 -- 220kV_Wesel_Ost_CN_24462426_220000_CN_24462228_220000/LConn1
  220kV_Dinslaken_West_CN_37554416_220000_CN_24462426_220000/RConn2 -- T_24462426_380000;220000;110000_Station_Niederrhein/RConn2 -- _CN_24462426_220000_CN_23084417_220000/LConn2 -- L_24462426/LConn2 -- 220kV_Scholven_E_CN_23022100_220000_CN_24462426_220000/RConn2 -- 220kV_Wesel_Ost_CN_24462426_220000_CN_23380800_220000/LConn2 -- 220kV_Wesel_Ost_CN_24462426_220000_CN_24462228_220000/LConn2
  220kV_Dinslaken_West_CN_37554416_220000_CN_24462426_220000/RConn3 -- T_24462426_380000;220000;110000_Station_Niederrhein/RConn3 -- _CN_24462426_220000_CN_23084417_220000/LConn3 -- L_24462426/LConn3 -- 220kV_Scholven_E_CN_23022100_220000_CN_24462426_220000/RConn3 -- 220kV_Wesel_Ost_CN_24462426_220000_CN_23380800_220000/LConn3 -- 220kV_Wesel_Ost_CN_24462426_220000_CN_24462228_220000/LConn3
  T_46852069_220000;110000_Station_Handbach/LConn1 -- 220kV_Dinslaken_West_CN_37554416_220000_CN_46852069_220000/RConn1
  T_46852069_220000;110000_Station_Handbach/LConn2 -- 220kV_Dinslaken_West_CN_37554416_220000_CN_46852069_220000/RConn2
  T_46852069_220000;110000_Station_Handbach/LConn3 -- 220kV_Dinslaken_West_CN_37554416_220000_CN_46852069_220000/RConn3
  220kV_Dinslaken_West_CN_37554416_220000_CN_24921206_220000/RConn1 -- T_24921206_380000;220000_Station_Büscherhof/RConn1 -- 220kV_LMG_West_CN_24921206_220000_CN_150267232_220000/LConn1 -- L_24921206/LConn1
  220kV_Dinslaken_West_CN_37554416_220000_CN_24921206_220000/RConn2 -- T_24921206_380000;220000_Station_Büscherhof/RConn2 -- 220kV_LMG_West_CN_24921206_220000_CN_150267232_220000/LConn2 -- L_24921206/LConn2
  220kV_Dinslaken_West_CN_37554416_220000_CN_24921206_220000/RConn3 -- T_24921206_380000;220000_Station_Büscherhof/RConn3 -- 220kV_LMG_West_CN_24921206_220000_CN_150267232_220000/LConn3 -- L_24921206/LConn3
  T_25032036_220000;110000_Styrum/LConn1 -- 220kV_Dinslaken_West_CN_37554416_220000_CN_25032036_220000/RConn1
  T_25032036_220000;110000_Styrum/LConn2 -- 220kV_Dinslaken_West_CN_37554416_220000_CN_25032036_220000/RConn2
  T_25032036_220000;110000_Styrum/LConn3 -- 220kV_Dinslaken_West_CN_37554416_220000_CN_25032036_220000/RConn3
  293_CN_137197826_220000_CN215092049/LConn1 -- T_137197826_380000;220000;110000_Neuenhagen/RConn1 -- L_137197826/LConn1
  293_CN_137197826_220000_CN215092049/LConn2 -- T_137197826_380000;220000;110000_Neuenhagen/RConn2 -- L_137197826/LConn2
  293_CN_137197826_220000_CN215092049/LConn3 -- T_137197826_380000;220000;110000_Neuenhagen/RConn3 -- L_137197826/LConn3
  293_CN_137197826_220000_CN215092049/RConn1 -- G_215092049_Solar_Energy_Field/RConn1 -- 294_CN_27149550_220000_CN215092049/LConn1 -- 306_CN_39437430_220000_CN215092049/LConn1
  293_CN_137197826_220000_CN215092049/RConn2 -- G_215092049_Solar_Energy_Field/RConn2 -- 294_CN_27149550_220000_CN215092049/LConn2 -- 306_CN_39437430_220000_CN215092049/LConn2
  293_CN_137197826_220000_CN215092049/RConn3 -- G_215092049_Solar_Energy_Field/RConn3 -- 294_CN_27149550_220000_CN215092049/LConn3 -- 306_CN_39437430_220000_CN215092049/LConn3
  548_CN_137197826_380000_CN_52983550_380000/LConn1 -- T_137197826_380000;220000;110000_Neuenhagen/LConn1 -- 517_CN_137197826_380000_CN_20562114_380000/LConn1 -- 495;_496_CN_137197826_380000_CN_22973070_380000/LConn1 -- 548_CN_137197826_380000_CN_23025610_380000/RConn1 -- 517_CN_137197826_380000_CN_29877599_380000/RConn1
  548_CN_137197826_380000_CN_52983550_380000/LConn2 -- T_137197826_380000;220000;110000_Neuenhagen/LConn2 -- 517_CN_137197826_380000_CN_20562114_380000/LConn2 -- 495;_496_CN_137197826_380000_CN_22973070_380000/LConn2 -- 548_CN_137197826_380000_CN_23025610_380000/RConn2 -- 517_CN_137197826_380000_CN_29877599_380000/RConn2
  548_CN_137197826_380000_CN_52983550_380000/LConn3 -- T_137197826_380000;220000;110000_Neuenhagen/LConn3 -- 517_CN_137197826_380000_CN_20562114_380000/LConn3 -- 495;_496_CN_137197826_380000_CN_22973070_380000/LConn3 -- 548_CN_137197826_380000_CN_23025610_380000/RConn3 -- 517_CN_137197826_380000_CN_29877599_380000/RConn3
  T_52983550_380000;110000_Eisenhüttenstadt/LConn1 -- 548_CN_137197826_380000_CN_52983550_380000/RConn1
  T_52983550_380000;110000_Eisenhüttenstadt/LConn2 -- 548_CN_137197826_380000_CN_52983550_380000/RConn2
  T_52983550_380000;110000_Eisenhüttenstadt/LConn3 -- 548_CN_137197826_380000_CN_52983550_380000/RConn3
  T_20562114_380000;110000_Umspannwerk_Malchow/LConn1 -- 517_CN_137197826_380000_CN_20562114_380000/RConn1
  T_20562114_380000;110000_Umspannwerk_Malchow/LConn2 -- 517_CN_137197826_380000_CN_20562114_380000/RConn2
  T_20562114_380000;110000_Umspannwerk_Malchow/LConn3 -- 517_CN_137197826_380000_CN_20562114_380000/RConn3
  495;_496_CN_137197826_380000_CN_22973070_380000/RConn1 -- T_22973070_380000;220000;110000_Umspannwerk_Marzahn/LConn1 -- _CN_22973070_380000_CN_30954714_380000/LConn1
  495;_496_CN_137197826_380000_CN_22973070_380000/RConn2 -- T_22973070_380000;220000;110000_Umspannwerk_Marzahn/LConn2 -- _CN_22973070_380000_CN_30954714_380000/LConn2
  495;_496_CN_137197826_380000_CN_22973070_380000/RConn3 -- T_22973070_380000;220000;110000_Umspannwerk_Marzahn/LConn3 -- _CN_22973070_380000_CN_30954714_380000/LConn3
  526_CN_29331499_220000_CN_27149550_220000/LConn1 -- T_29331499_380000;220000;110000_Thyrow/RConn1 -- 302_CN_29331499_220000_CN_22973070_220000/LConn1 -- 302_CN_29331499_220000_CN_22973052_220000/LConn1 -- L_29331499/LConn1
  526_CN_29331499_220000_CN_27149550_220000/LConn2 -- T_29331499_380000;220000;110000_Thyrow/RConn2 -- 302_CN_29331499_220000_CN_22973070_220000/LConn2 -- 302_CN_29331499_220000_CN_22973052_220000/LConn2 -- L_29331499/LConn2
  526_CN_29331499_220000_CN_27149550_220000/LConn3 -- T_29331499_380000;220000;110000_Thyrow/RConn3 -- 302_CN_29331499_220000_CN_22973070_220000/LConn3 -- 302_CN_29331499_220000_CN_22973052_220000/LConn3 -- L_29331499/LConn3
  526_CN_29331499_220000_CN_27149550_220000/RConn1 -- T_27149550_380000;220000;110000_Wustermark/RConn1 -- 294_CN_27149550_220000_CN215092049/RConn1 -- 294_CN_27149550_220000_CN_30309989_220000/LConn1 -- L_27149550/LConn1 -- 324_CN_40621568_220000_CN_27149550_220000/LConn1
  526_CN_29331499_220000_CN_27149550_220000/RConn2 -- T_27149550_380000;220000;110000_Wustermark/RConn2 -- 294_CN_27149550_220000_CN215092049/RConn2 -- 294_CN_27149550_220000_CN_30309989_220000/LConn2 -- L_27149550/LConn2 -- 324_CN_40621568_220000_CN_27149550_220000/LConn2
  526_CN_29331499_220000_CN_27149550_220000/RConn3 -- T_27149550_380000;220000;110000_Wustermark/RConn3 -- 294_CN_27149550_220000_CN215092049/RConn3 -- 294_CN_27149550_220000_CN_30309989_220000/LConn3 -- L_27149550/LConn3 -- 324_CN_40621568_220000_CN_27149550_220000/LConn3
  302_CN_29331499_220000_CN_22973070_220000/RConn1 -- T_22973070_380000;220000;110000_Umspannwerk_Marzahn/RConn1 -- L_22973070/LConn1
  302_CN_29331499_220000_CN_22973070_220000/RConn2 -- T_22973070_380000;220000;110000_Umspannwerk_Marzahn/RConn2 -- L_22973070/LConn2
  302_CN_29331499_220000_CN_22973070_220000/RConn3 -- T_22973070_380000;220000;110000_Umspannwerk_Marzahn/RConn3 -- L_22973070/LConn3
  T_22973052_220000;110000_Umspannwerk_Wuhlheide/LConn1 -- 302_CN_29331499_220000_CN_22973052_220000/RConn1
  T_22973052_220000;110000_Umspannwerk_Wuhlheide/LConn2 -- 302_CN_29331499_220000_CN_22973052_220000/RConn2
  T_22973052_220000;110000_Umspannwerk_Wuhlheide/LConn3 -- 302_CN_29331499_220000_CN_22973052_220000/RConn3
  T_29331499_380000;220000;110000_Thyrow/LConn1 -- 522_CN_29331499_380000_CN_27149550_380000/LConn1
  T_29331499_380000;220000;110000_Thyrow/LConn2 -- 522_CN_29331499_380000_CN_27149550_380000/LConn2
  T_29331499_380000;220000;110000_Thyrow/LConn3 -- 522_CN_29331499_380000_CN_27149550_380000/LConn3
  522_CN_29331499_380000_CN_27149550_380000/RConn1 -- T_27149550_380000;220000;110000_Wustermark/LConn1 -- 493_CN_26472665_380000_CN_27149550_380000/LConn1
  522_CN_29331499_380000_CN_27149550_380000/RConn2 -- T_27149550_380000;220000;110000_Wustermark/LConn2 -- 493_CN_26472665_380000_CN_27149550_380000/LConn2
  522_CN_29331499_380000_CN_27149550_380000/RConn3 -- T_27149550_380000;220000;110000_Wustermark/LConn3 -- 493_CN_26472665_380000_CN_27149550_380000/LConn3
  Helmstedt_380_kV_CN_26474759_380000_CN_24258096_380000/RConn1 -- T_26474759_380000;110000_Umspannwerk_Helmstedt/LConn1 -- Helmstedt_380_kV_CN_26474759_380000_CN_26472665_380000/LConn1 -- Leitung_3845_(System_301)_CN_26474759_380000_CN237147926/LConn1
  Helmstedt_380_kV_CN_26474759_380000_CN_24258096_380000/RConn2 -- T_26474759_380000;110000_Umspannwerk_Helmstedt/LConn2 -- Helmstedt_380_kV_CN_26474759_380000_CN_26472665_380000/LConn2 -- Leitung_3845_(System_301)_CN_26474759_380000_CN237147926/LConn2
  Helmstedt_380_kV_CN_26474759_380000_CN_24258096_380000/RConn3 -- T_26474759_380000;110000_Umspannwerk_Helmstedt/LConn3 -- Helmstedt_380_kV_CN_26474759_380000_CN_26472665_380000/LConn3 -- Leitung_3845_(System_301)_CN_26474759_380000_CN237147926/LConn3
  G_237147926_Kraftwerk_Buschhaus/RConn1 -- Leitung_3845_(System_301)_CN_26474759_380000_CN237147926/RConn1
  G_237147926_Kraftwerk_Buschhaus/RConn2 -- Leitung_3845_(System_301)_CN_26474759_380000_CN237147926/RConn2
  G_237147926_Kraftwerk_Buschhaus/RConn3 -- Leitung_3845_(System_301)_CN_26474759_380000_CN237147926/RConn3
  Helmstedt_380_kV_CN_26474759_380000_CN_26472665_380000/RConn1 -- T_26472665_380000;220000_Umspannwerk_Wolmirstedt/LConn1 -- 493_CN_26472665_380000_CN_30132758_380000/LConn1 -- 493_CN_26472665_380000_CN_27149550_380000/RConn1 -- 438_CN_26472665_380000_CN_156683994_380000/LConn1 -- 536_CN_26472665_380000_CN_32690742_380000/LConn1 -- 536_CN_26472665_380000_CN_29713902_380000/LConn1 -- 490_CN_26472665_380000_CN_33169401_380000/RConn1
  Helmstedt_380_kV_CN_26474759_380000_CN_26472665_380000/RConn2 -- T_26472665_380000;220000_Umspannwerk_Wolmirstedt/LConn2 -- 493_CN_26472665_380000_CN_30132758_380000/LConn2 -- 493_CN_26472665_380000_CN_27149550_380000/RConn2 -- 438_CN_26472665_380000_CN_156683994_380000/LConn2 -- 536_CN_26472665_380000_CN_32690742_380000/LConn2 -- 536_CN_26472665_380000_CN_29713902_380000/LConn2 -- 490_CN_26472665_380000_CN_33169401_380000/RConn2
  Helmstedt_380_kV_CN_26474759_380000_CN_26472665_380000/RConn3 -- T_26472665_380000;220000_Umspannwerk_Wolmirstedt/LConn3 -- 493_CN_26472665_380000_CN_30132758_380000/LConn3 -- 493_CN_26472665_380000_CN_27149550_380000/RConn3 -- 438_CN_26472665_380000_CN_156683994_380000/LConn3 -- 536_CN_26472665_380000_CN_32690742_380000/LConn3 -- 536_CN_26472665_380000_CN_29713902_380000/LConn3 -- 490_CN_26472665_380000_CN_33169401_380000/RConn3
  _CN_29344008_220000_CN_151765495_220000/RConn1 -- T_151765495_220000_Götzdorf/LConn1 -- _CN_151765495_220000_CN_229500139_220000/LConn1
  _CN_29344008_220000_CN_151765495_220000/RConn2 -- T_151765495_220000_Götzdorf/LConn2 -- _CN_151765495_220000_CN_229500139_220000/LConn2
  _CN_29344008_220000_CN_151765495_220000/RConn3 -- T_151765495_220000_Götzdorf/LConn3 -- _CN_151765495_220000_CN_229500139_220000/LConn3
  T_25306938_220000;110000_Kummerfeld/LConn1 -- _CN_29344008_220000_CN_25306938_220000/RConn1
  T_25306938_220000;110000_Kummerfeld/LConn2 -- _CN_29344008_220000_CN_25306938_220000/RConn2
  T_25306938_220000;110000_Kummerfeld/LConn3 -- _CN_29344008_220000_CN_25306938_220000/RConn3
  T_167352587_220000;110000_Umspannwerk_Herlasgrün/LConn1 -- 231;_232_Weida___Herlasgrün_CN_167352587_220000_CN_156673637_220000/LConn1
  T_167352587_220000;110000_Umspannwerk_Herlasgrün/LConn2 -- 231;_232_Weida___Herlasgrün_CN_167352587_220000_CN_156673637_220000/LConn2
  T_167352587_220000;110000_Umspannwerk_Herlasgrün/LConn3 -- 231;_232_Weida___Herlasgrün_CN_167352587_220000_CN_156673637_220000/LConn3
  231;_232_Weida___Herlasgrün_CN_167352587_220000_CN_156673637_220000/RConn1 -- T_156673637_380000;220000;110000_Umspannwerk_Weida/RConn1 -- L_156673637/LConn1
  231;_232_Weida___Herlasgrün_CN_167352587_220000_CN_156673637_220000/RConn2 -- T_156673637_380000;220000;110000_Umspannwerk_Weida/RConn2 -- L_156673637/LConn2
  231;_232_Weida___Herlasgrün_CN_167352587_220000_CN_156673637_220000/RConn3 -- T_156673637_380000;220000;110000_Umspannwerk_Weida/RConn3 -- L_156673637/LConn3
  T_169244940_380000_Station_Kelsterbach/LConn1 -- _CN_169244940_380000_CN_55730023_380000/LConn1
  T_169244940_380000_Station_Kelsterbach/LConn2 -- _CN_169244940_380000_CN_55730023_380000/LConn2
  T_169244940_380000_Station_Kelsterbach/LConn3 -- _CN_169244940_380000_CN_55730023_380000/LConn3
  _CN_169244940_380000_CN_55730023_380000/RConn1 -- T_55730023_380000_Kabeleinführung_380_kV/LConn1 -- 2_x_380_kV;_3_x_220_kV_CN_23284340_380000_CN_55730023_380000/LConn1
  _CN_169244940_380000_CN_55730023_380000/RConn2 -- T_55730023_380000_Kabeleinführung_380_kV/LConn2 -- 2_x_380_kV;_3_x_220_kV_CN_23284340_380000_CN_55730023_380000/LConn2
  _CN_169244940_380000_CN_55730023_380000/RConn3 -- T_55730023_380000_Kabeleinführung_380_kV/LConn3 -- 2_x_380_kV;_3_x_220_kV_CN_23284340_380000_CN_55730023_380000/LConn3
  T_29417741_220000_Umspannwerk_Regensburg/LConn1 -- Regensburg___Schwandorf_CN_29417741_220000_CN_28956649_220000/LConn1
  T_29417741_220000_Umspannwerk_Regensburg/LConn2 -- Regensburg___Schwandorf_CN_29417741_220000_CN_28956649_220000/LConn2
  T_29417741_220000_Umspannwerk_Regensburg/LConn3 -- Regensburg___Schwandorf_CN_29417741_220000_CN_28956649_220000/LConn3
  Regensburg___Schwandorf_CN_29417741_220000_CN_28956649_220000/RConn1 -- T_28956649_380000;220000;110000_Schwandorf/RConn1 -- Ludersheim___Schwandorf_CN_133349218_220000_CN_28956649_220000/LConn1 -- L_28956649/LConn1 -- Pleinting___Schwandorf_CN_24976300_220000_CN_28956649_220000/LConn1 -- MH___SD_CN_93341407_220000_CN_28956649_220000/LConn1
  Regensburg___Schwandorf_CN_29417741_220000_CN_28956649_220000/RConn2 -- T_28956649_380000;220000;110000_Schwandorf/RConn2 -- Ludersheim___Schwandorf_CN_133349218_220000_CN_28956649_220000/LConn2 -- L_28956649/LConn2 -- Pleinting___Schwandorf_CN_24976300_220000_CN_28956649_220000/LConn2 -- MH___SD_CN_93341407_220000_CN_28956649_220000/LConn2
  Regensburg___Schwandorf_CN_29417741_220000_CN_28956649_220000/RConn3 -- T_28956649_380000;220000;110000_Schwandorf/RConn3 -- Ludersheim___Schwandorf_CN_133349218_220000_CN_28956649_220000/LConn3 -- L_28956649/LConn3 -- Pleinting___Schwandorf_CN_24976300_220000_CN_28956649_220000/LConn3 -- MH___SD_CN_93341407_220000_CN_28956649_220000/LConn3
  _CN_145002769_380000_CN_143903369_380000/LConn1 -- T_145002769_380000;110000_Umspannwerk_Höpfingen/LConn1 -- _CN_145002769_380000_CN_108797675_380000/RConn1 -- _CN_145002769_380000_CN_143854536_380000/LConn1 -- _CN_145002769_380000_CN_25557397_380000/LConn1
  _CN_145002769_380000_CN_143903369_380000/LConn2 -- T_145002769_380000;110000_Umspannwerk_Höpfingen/LConn2 -- _CN_145002769_380000_CN_108797675_380000/RConn2 -- _CN_145002769_380000_CN_143854536_380000/LConn2 -- _CN_145002769_380000_CN_25557397_380000/LConn2
  _CN_145002769_380000_CN_143903369_380000/LConn3 -- T_145002769_380000;110000_Umspannwerk_Höpfingen/LConn3 -- _CN_145002769_380000_CN_108797675_380000/RConn3 -- _CN_145002769_380000_CN_143854536_380000/LConn3 -- _CN_145002769_380000_CN_25557397_380000/LConn3
  _CN_145002769_380000_CN_143903369_380000/RConn1 -- T_143903369_380000;220000;110000_Umspannwerk_Hüffenhardt/LConn1 -- Elsenz_CN_143903369_380000_CN_46584363_380000/LConn1 -- Elsenz_CN_143903369_380000_CN161909939/RConn1 -- Elsenz_CN_143903369_380000_CN_207248812_380000/LConn1
  _CN_145002769_380000_CN_143903369_380000/RConn2 -- T_143903369_380000;220000;110000_Umspannwerk_Hüffenhardt/LConn2 -- Elsenz_CN_143903369_380000_CN_46584363_380000/LConn2 -- Elsenz_CN_143903369_380000_CN161909939/RConn2 -- Elsenz_CN_143903369_380000_CN_207248812_380000/LConn2
  _CN_145002769_380000_CN_143903369_380000/RConn3 -- T_143903369_380000;220000;110000_Umspannwerk_Hüffenhardt/LConn3 -- Elsenz_CN_143903369_380000_CN_46584363_380000/LConn3 -- Elsenz_CN_143903369_380000_CN161909939/RConn3 -- Elsenz_CN_143903369_380000_CN_207248812_380000/LConn3
  _CN_145002769_380000_CN_25557397_380000/RConn1 -- T_25557397_380000;220000;110000_380_kV_Umspannwerk_Großgartach/LConn1 -- _CN_25557397_380000_CN_43688805_380000/LConn1 -- _CN_25557397_380000_CN89183108/LConn1 -- _CN_25557397_380000_CN_143854536_380000/LConn1 -- _CN_25557397_380000_CN23547196/RConn1
  _CN_145002769_380000_CN_25557397_380000/RConn2 -- T_25557397_380000;220000;110000_380_kV_Umspannwerk_Großgartach/LConn2 -- _CN_25557397_380000_CN_43688805_380000/LConn2 -- _CN_25557397_380000_CN89183108/LConn2 -- _CN_25557397_380000_CN_143854536_380000/LConn2 -- _CN_25557397_380000_CN23547196/RConn2
  _CN_145002769_380000_CN_25557397_380000/RConn3 -- T_25557397_380000;220000;110000_380_kV_Umspannwerk_Großgartach/LConn3 -- _CN_25557397_380000_CN_43688805_380000/LConn3 -- _CN_25557397_380000_CN89183108/LConn3 -- _CN_25557397_380000_CN_143854536_380000/LConn3 -- _CN_25557397_380000_CN23547196/RConn3
  _CN_145002769_380000_CN_143854536_380000/RConn1 -- T_143854536_380000;110000_Umspannwerk_Kupferzell/LConn1 -- _CN_25557397_380000_CN_143854536_380000/RConn1 -- Goldshöfe___Kupferzell_CN_42050342_380000_CN_143854536_380000/RConn1
  _CN_145002769_380000_CN_143854536_380000/RConn2 -- T_143854536_380000;110000_Umspannwerk_Kupferzell/LConn2 -- _CN_25557397_380000_CN_143854536_380000/RConn2 -- Goldshöfe___Kupferzell_CN_42050342_380000_CN_143854536_380000/RConn2
  _CN_145002769_380000_CN_143854536_380000/RConn3 -- T_143854536_380000;110000_Umspannwerk_Kupferzell/LConn3 -- _CN_25557397_380000_CN_143854536_380000/RConn3 -- Goldshöfe___Kupferzell_CN_42050342_380000_CN_143854536_380000/RConn3
  501_CN_28729619_380000_CN_25526912_380000/LConn1 -- T_28729619_380000_Umspannwerk_Schönewalde/LConn1 -- 501_CN_28729619_380000_CN_156683994_380000/LConn1 -- 501_CN_28729619_380000_CN_29713902_380000/LConn1
  501_CN_28729619_380000_CN_25526912_380000/LConn2 -- T_28729619_380000_Umspannwerk_Schönewalde/LConn2 -- 501_CN_28729619_380000_CN_156683994_380000/LConn2 -- 501_CN_28729619_380000_CN_29713902_380000/LConn2
  501_CN_28729619_380000_CN_25526912_380000/LConn3 -- T_28729619_380000_Umspannwerk_Schönewalde/LConn3 -- 501_CN_28729619_380000_CN_156683994_380000/LConn3 -- 501_CN_28729619_380000_CN_29713902_380000/LConn3
  T_25526912_380000;110000_Umspannwerk_Marke/LConn1 -- 501_CN_28729619_380000_CN_25526912_380000/RConn1
  T_25526912_380000;110000_Umspannwerk_Marke/LConn2 -- 501_CN_28729619_380000_CN_25526912_380000/RConn2
  T_25526912_380000;110000_Umspannwerk_Marke/LConn3 -- 501_CN_28729619_380000_CN_25526912_380000/RConn3
  501_CN_28729619_380000_CN_29713902_380000/RConn1 -- T_29713902_380000;110000_Umspannwerk_Lauchstädt/LConn1 -- _CN_29713902_380000_CN218161891/LConn1 -- _CN_143882655_380000_CN_29713902_380000/RConn1 -- 536_CN_26472665_380000_CN_29713902_380000/RConn1
  501_CN_28729619_380000_CN_29713902_380000/RConn2 -- T_29713902_380000;110000_Umspannwerk_Lauchstädt/LConn2 -- _CN_29713902_380000_CN218161891/LConn2 -- _CN_143882655_380000_CN_29713902_380000/RConn2 -- 536_CN_26472665_380000_CN_29713902_380000/RConn2
  501_CN_28729619_380000_CN_29713902_380000/RConn3 -- T_29713902_380000;110000_Umspannwerk_Lauchstädt/LConn3 -- _CN_29713902_380000_CN218161891/LConn3 -- _CN_143882655_380000_CN_29713902_380000/RConn3 -- 536_CN_26472665_380000_CN_29713902_380000/RConn3
  501_CN_28729619_380000_CN_156683994_380000/RConn1 -- T_156683994_380000;110000_Umspannwerk_Ragow/LConn1 -- _CN_156683994_380000_CN_23025610_380000/RConn1 -- 438_CN_26472665_380000_CN_156683994_380000/RConn1 -- 561_Streumen_CN_156683994_380000_CN_157328339_380000/LConn1
  501_CN_28729619_380000_CN_156683994_380000/RConn2 -- T_156683994_380000;110000_Umspannwerk_Ragow/LConn2 -- _CN_156683994_380000_CN_23025610_380000/RConn2 -- 438_CN_26472665_380000_CN_156683994_380000/RConn2 -- 561_Streumen_CN_156683994_380000_CN_157328339_380000/LConn2
  501_CN_28729619_380000_CN_156683994_380000/RConn3 -- T_156683994_380000;110000_Umspannwerk_Ragow/LConn3 -- _CN_156683994_380000_CN_23025610_380000/RConn3 -- 438_CN_26472665_380000_CN_156683994_380000/RConn3 -- 561_Streumen_CN_156683994_380000_CN_157328339_380000/LConn3
  T_53378027_380000;110000_Umspannwerk_Lechhausen;_Übernahmestation_Lechhausen/LConn1 -- _CN_30613895_380000_CN_53378027_380000/RConn1
  T_53378027_380000;110000_Umspannwerk_Lechhausen;_Übernahmestation_Lechhausen/LConn2 -- _CN_30613895_380000_CN_53378027_380000/RConn2
  T_53378027_380000;110000_Umspannwerk_Lechhausen;_Übernahmestation_Lechhausen/LConn3 -- _CN_30613895_380000_CN_53378027_380000/RConn3
  _CN_30613895_380000_CN_24652261_380000/RConn1 -- T_24652261_380000_Station_Meitingen/LConn1 -- Meitingen_Nord;_Süd_CN_24652261_380000_CN_85523877_380000/RConn1 -- Meitingen_Nord;_Süd_CN_24652261_380000_CN_88945213_380000/LConn1 -- _CN_24652261_380000_CN_76246159_380000/LConn1 -- MEI_OBA_CN_24652261_380000_CN_18629425_380000/RConn1
  _CN_30613895_380000_CN_24652261_380000/RConn2 -- T_24652261_380000_Station_Meitingen/LConn2 -- Meitingen_Nord;_Süd_CN_24652261_380000_CN_85523877_380000/RConn2 -- Meitingen_Nord;_Süd_CN_24652261_380000_CN_88945213_380000/LConn2 -- _CN_24652261_380000_CN_76246159_380000/LConn2 -- MEI_OBA_CN_24652261_380000_CN_18629425_380000/RConn2
  _CN_30613895_380000_CN_24652261_380000/RConn3 -- T_24652261_380000_Station_Meitingen/LConn3 -- Meitingen_Nord;_Süd_CN_24652261_380000_CN_85523877_380000/RConn3 -- Meitingen_Nord;_Süd_CN_24652261_380000_CN_88945213_380000/LConn3 -- _CN_24652261_380000_CN_76246159_380000/LConn3 -- MEI_OBA_CN_24652261_380000_CN_18629425_380000/RConn3
  305_CN_35176751_380000_CN_301158539_380000/LConn1 -- T_35176751_380000;110000_Audorf/LConn1 -- 305_CN_35176751_380000_CN_87952821_380000/LConn1 -- 303_CN_35176751_380000_CN_28502915_380000/RConn1
  305_CN_35176751_380000_CN_301158539_380000/LConn2 -- T_35176751_380000;110000_Audorf/LConn2 -- 305_CN_35176751_380000_CN_87952821_380000/LConn2 -- 303_CN_35176751_380000_CN_28502915_380000/RConn2
  305_CN_35176751_380000_CN_301158539_380000/LConn3 -- T_35176751_380000;110000_Audorf/LConn3 -- 305_CN_35176751_380000_CN_87952821_380000/LConn3 -- 303_CN_35176751_380000_CN_28502915_380000/RConn3
  T_301158539_380000;110000;20000_Umspannwerk_Jardelund/LConn1 -- 305_CN_35176751_380000_CN_301158539_380000/RConn1
  T_301158539_380000;110000;20000_Umspannwerk_Jardelund/LConn2 -- 305_CN_35176751_380000_CN_301158539_380000/RConn2
  T_301158539_380000;110000;20000_Umspannwerk_Jardelund/LConn3 -- 305_CN_35176751_380000_CN_301158539_380000/RConn3
  T_87952821_380000;220000;110000;20000_Flensburg/LConn1 -- 305_CN_35176751_380000_CN_87952821_380000/RConn1
  T_87952821_380000;220000;110000;20000_Flensburg/LConn2 -- 305_CN_35176751_380000_CN_87952821_380000/RConn2
  T_87952821_380000;220000;110000;20000_Flensburg/LConn3 -- 305_CN_35176751_380000_CN_87952821_380000/RConn3
  220kV_Welper_Ost+ANK_CN_156973363_220000_CN_63114179_220000/LConn1 -- T_156973363_220000_Station_Welper/LConn1 -- 220kV_Welper_Ost+ANK_CN_156973363_220000_CN_86163350_220000/LConn1 -- 220kV_Welper_Ost+ANK_CN_156973363_220000_CN_68549340_220000/RConn1
  220kV_Welper_Ost+ANK_CN_156973363_220000_CN_63114179_220000/LConn2 -- T_156973363_220000_Station_Welper/LConn2 -- 220kV_Welper_Ost+ANK_CN_156973363_220000_CN_86163350_220000/LConn2 -- 220kV_Welper_Ost+ANK_CN_156973363_220000_CN_68549340_220000/RConn2
  220kV_Welper_Ost+ANK_CN_156973363_220000_CN_63114179_220000/LConn3 -- T_156973363_220000_Station_Welper/LConn3 -- 220kV_Welper_Ost+ANK_CN_156973363_220000_CN_86163350_220000/LConn3 -- 220kV_Welper_Ost+ANK_CN_156973363_220000_CN_68549340_220000/RConn3
  220kV_Welper_Ost+ANK_CN_156973363_220000_CN_63114179_220000/RConn1 -- T_63114179_380000;220000;110000_Station_Hattingen/RConn1 -- L_63114179/LConn1
  220kV_Welper_Ost+ANK_CN_156973363_220000_CN_63114179_220000/RConn2 -- T_63114179_380000;220000;110000_Station_Hattingen/RConn2 -- L_63114179/LConn2
  220kV_Welper_Ost+ANK_CN_156973363_220000_CN_63114179_220000/RConn3 -- T_63114179_380000;220000;110000_Station_Hattingen/RConn3 -- L_63114179/LConn3
  T_86163350_220000_UW_Stahlwerk_ThyssenKrupp_Nirosta/LConn1 -- 220kV_Welper_Ost+ANK_CN_156973363_220000_CN_86163350_220000/RConn1
  T_86163350_220000_UW_Stahlwerk_ThyssenKrupp_Nirosta/LConn2 -- 220kV_Welper_Ost+ANK_CN_156973363_220000_CN_86163350_220000/RConn2
  T_86163350_220000_UW_Stahlwerk_ThyssenKrupp_Nirosta/LConn3 -- 220kV_Welper_Ost+ANK_CN_156973363_220000_CN_86163350_220000/RConn3
  ETZ___MH___RED_CN_93341407_380000_CN_29084374_380000/LConn1 -- T_93341407_380000;220000;110000_Umspannwerk_Mechlenreuth/LConn1 -- Etzenricht___Mechlenreuth___Redwitz_CN_93341407_380000_CN_24757392_380000/RConn1
  ETZ___MH___RED_CN_93341407_380000_CN_29084374_380000/LConn2 -- T_93341407_380000;220000;110000_Umspannwerk_Mechlenreuth/LConn2 -- Etzenricht___Mechlenreuth___Redwitz_CN_93341407_380000_CN_24757392_380000/RConn2
  ETZ___MH___RED_CN_93341407_380000_CN_29084374_380000/LConn3 -- T_93341407_380000;220000;110000_Umspannwerk_Mechlenreuth/LConn3 -- Etzenricht___Mechlenreuth___Redwitz_CN_93341407_380000_CN_24757392_380000/RConn3
  ETZ___MH___RED_CN_93341407_380000_CN_29084374_380000/RConn1 -- T_29084374_380000;110000_Umspannwerk_Etzenricht/LConn1 -- Schwandorf___Etzenricht_CN_29084374_380000_CN_28956649_380000/LConn1
  ETZ___MH___RED_CN_93341407_380000_CN_29084374_380000/RConn2 -- T_29084374_380000;110000_Umspannwerk_Etzenricht/LConn2 -- Schwandorf___Etzenricht_CN_29084374_380000_CN_28956649_380000/LConn2
  ETZ___MH___RED_CN_93341407_380000_CN_29084374_380000/RConn3 -- T_29084374_380000;110000_Umspannwerk_Etzenricht/LConn3 -- Schwandorf___Etzenricht_CN_29084374_380000_CN_28956649_380000/LConn3
  MH___SD_CN_93341407_220000_CN_28956649_220000/RConn1 -- T_93341407_380000;220000;110000_Umspannwerk_Mechlenreuth/RConn1 -- L_93341407/LConn1
  MH___SD_CN_93341407_220000_CN_28956649_220000/RConn2 -- T_93341407_380000;220000;110000_Umspannwerk_Mechlenreuth/RConn2 -- L_93341407/LConn2
  MH___SD_CN_93341407_220000_CN_28956649_220000/RConn3 -- T_93341407_380000;220000;110000_Umspannwerk_Mechlenreuth/RConn3 -- L_93341407/LConn3
  329_CN_35102433_220000_CN_26472665_220000/LConn1 -- T_35102433_220000;110000_Magdeburg_(50Hertz)/LConn1 -- 335_CN_35102433_220000_CN_35137205_220000/LConn1
  329_CN_35102433_220000_CN_26472665_220000/LConn2 -- T_35102433_220000;110000_Magdeburg_(50Hertz)/LConn2 -- 335_CN_35102433_220000_CN_35137205_220000/LConn2
  329_CN_35102433_220000_CN_26472665_220000/LConn3 -- T_35102433_220000;110000_Magdeburg_(50Hertz)/LConn3 -- 335_CN_35102433_220000_CN_35137205_220000/LConn3
  329_CN_35102433_220000_CN_26472665_220000/RConn1 -- T_26472665_380000;220000_Umspannwerk_Wolmirstedt/RConn1 -- 344_CN_26472665_220000_CN_35137205_220000/LConn1 -- L_26472665/LConn1
  329_CN_35102433_220000_CN_26472665_220000/RConn2 -- T_26472665_380000;220000_Umspannwerk_Wolmirstedt/RConn2 -- 344_CN_26472665_220000_CN_35137205_220000/LConn2 -- L_26472665/LConn2
  329_CN_35102433_220000_CN_26472665_220000/RConn3 -- T_26472665_380000;220000_Umspannwerk_Wolmirstedt/RConn3 -- 344_CN_26472665_220000_CN_35137205_220000/LConn3 -- L_26472665/LConn3
  335_CN_35102433_220000_CN_35137205_220000/RConn1 -- T_35137205_220000;110000_Umspannwerk_Förderstedt/LConn1 -- 344_CN_26472665_220000_CN_35137205_220000/RConn1
  335_CN_35102433_220000_CN_35137205_220000/RConn2 -- T_35137205_220000;110000_Umspannwerk_Förderstedt/LConn2 -- 344_CN_26472665_220000_CN_35137205_220000/RConn2
  335_CN_35102433_220000_CN_35137205_220000/RConn3 -- T_35137205_220000;110000_Umspannwerk_Förderstedt/LConn3 -- 344_CN_26472665_220000_CN_35137205_220000/RConn3
  _CN_91086220_220000_CN_24976300_220000/LConn1 -- T_91086220_220000_Umspannwerk_Simbach/LConn1 -- _CN_91086220_220000_CN_77694901_220000/LConn1 -- _CN_91086220_220000_CN167578660/RConn1
  _CN_91086220_220000_CN_24976300_220000/LConn2 -- T_91086220_220000_Umspannwerk_Simbach/LConn2 -- _CN_91086220_220000_CN_77694901_220000/LConn2 -- _CN_91086220_220000_CN167578660/RConn2
  _CN_91086220_220000_CN_24976300_220000/LConn3 -- T_91086220_220000_Umspannwerk_Simbach/LConn3 -- _CN_91086220_220000_CN_77694901_220000/LConn3 -- _CN_91086220_220000_CN167578660/RConn3
  _CN_91086220_220000_CN_24976300_220000/RConn1 -- T_24976300_380000;220000;110000_Umspannwerk_Pleinting/RConn1 -- Pleinting___Schwandorf_CN_24976300_220000_CN_28956649_220000/RConn1 -- L_24976300/LConn1
  _CN_91086220_220000_CN_24976300_220000/RConn2 -- T_24976300_380000;220000;110000_Umspannwerk_Pleinting/RConn2 -- Pleinting___Schwandorf_CN_24976300_220000_CN_28956649_220000/RConn2 -- L_24976300/LConn2
